simulink library "outp"  (R2021b)
settings: Solver=VariableStepAuto  StartTime=0.0  StopTime=10.0  RelTol=1e-3
undefined symbols (not defined in the file or in its folder): ENUM_PMMMODE_CHARGE, ENUM_PMMMODE_IDLE, ENUM_PMMMODE_INITIALIZE, ENUM_PMMMODE_POWERDOWN, ENUM_PMMMODE_SLEEP, Left, outp, slcm, TRUE
libraries: FVT_lib x736, hcu_lib x4, simulink x1
(part 4 of 8)

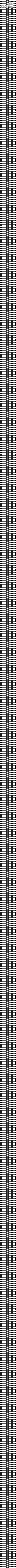
== system outp/OUTP/outpmodule ==
  VACC_HVTHCMSysAvail_enum : Inport
  VACC_LVBattVoltSta_enum : Inport  Port=2
  VACC_VehHVPwrAvail4THCM_W : Inport  Port=3
  VAPM_VehSpeed_kph : Inport  Port=4
  VAPM_VehSpeedTimeOut_flg : Inport  Port=5
  VAPM_FSOffSw_enum : Inport  Port=6
  VAPM_FSOffSwTimeOut_flg : Inport  Port=7
  VAPM_ChrgPlugSta_enum : Inport  Port=8
  VAPM_PASDRMR_cm : Inport  Port=9
  VAPM_PASDRML_cm : Inport  Port=10
  VAPM_PASDRCR_cm : Inport  Port=11
  VAPM_PASDRCL_cm : Inport  Port=12
  VAPM_PASDFMR_cm : Inport  Port=13
  VAPM_PASDFML_cm : Inport  Port=14
  VAPM_PASDFCR_cm : Inport  Port=15
  VAPM_PASDFCL_cm : Inport  Port=16
  VAPM_APSDRLR_cm : Inport  Port=17
  VAPM_APSDRLL_cm : Inport  Port=18
  VAPM_APSDFLR_cm : Inport  Port=19
  VAPM_APSDFLL_cm : Inport  Port=20
  VAPM_PASAFCL_enum : Inport  Port=21
  VAPM_PASARMR_enum : Inport  Port=22
  VAPM_PASARML_enum : Inport  Port=23
  VAPM_PASARCR_enum : Inport  Port=24
  VAPM_PASARCL_enum : Inport  Port=25
  VAPM_PASAFMR_enum : Inport  Port=26
  VAPM_PASAFML_enum : Inport  Port=27
  VAPM_PASAFCR_enum : Inport  Port=28
  VAPM_USSStaRMR_flg : Inport  Port=29
  VAPM_USSStaRML_flg : Inport  Port=30
  VAPM_USSStaRLR_flg : Inport  Port=31
  VAPM_USSStaRLL_flg : Inport  Port=32
  VAPM_USSStaRCR_flg : Inport  Port=33
  VAPM_USSStaRCL_flg : Inport  Port=34
  VAPM_USSStaFMR_flg : Inport  Port=35
  VAPM_USSStaFML_flg : Inport  Port=36
  VAPM_USSStaFLR_flg : Inport  Port=37
  VAPM_USSStaFLL_flg : Inport  Port=38
  VAPM_USSStaFCR_flg : Inport  Port=39
  VAPM_USSStaFCL_flg : Inport  Port=40
  VAPM_Chime_enum : Inport  Port=41
  VAPM_SNSRLayout_enum : Inport  Port=42
  VAPM_StaFSya_flg : Inport  Port=43
  VAPM_ModOperation_enum : Inport  Port=44
  VAPM_BrkPedalPos_pct : Inport  Port=45
  VAPM_BrkPedalPosTimeOut_flg : Inport  Port=46
  VAPM_LFRawWhlSpeed_kph : Inport  Port=47
  VAPM_LFRawWhlSpeedTimeOut_flg : Inport  Port=48
  VAPM_RFRawWhlSpeed_kph : Inport  Port=49
  VAPM_RFRawWhlSpeedTimeOut_flg : Inport  Port=50
  VAPM_LRRawWhlSpeed_kph : Inport  Port=51
  VAPM_LRRawWhlSpeedTimeOut_flg : Inport  Port=52
  VAPM_RRRawWhlSpeed_kph : Inport  Port=53
  VAPM_RRRawWhlSpeedTimeOut_flg : Inport  Port=54
  VAPM_LFRawWhlSpeedV_flg : Inport  Port=55
  VAPM_LFRawWhlSpeedVTimeOut_flg : Inport  Port=56
  VAPM_RFRawWhlSpeedV_flg : Inport  Port=57
  VAPM_RFRawWhlSpeedVTimeOut_flg : Inport  Port=58
  VAPM_LRRawWhlSpeedV_flg : Inport  Port=59
  VAPM_LRRawWhlSpeedVTimeOut_flg : Inport  Port=60
  VAPM_RRRawWhlSpeedV_flg : Inport  Port=61
  VAPM_RRRawWhlSpeedVTimeOut_flg : Inport  Port=62
  VAPM_LFWhlRotDir_enum : Inport  Port=63
  VAPM_LFWhlRotDirTimeOut_flg : Inport  Port=64
  VAPM_RFWhlRotDir_enum : Inport  Port=65
  VAPM_RFWhlRotDirTimeOut_flg : Inport  Port=66
  VAPM_LRWhlRotDir_enum : Inport  Port=67
  VAPM_LRWhlRotDirTimeOut_flg : Inport  Port=68
  VAPM_RRWhlRotDir_enum : Inport  Port=69
  VAPM_RRWhlRotDirTimeOut_flg : Inport  Port=70
  VAPM_LFPulseCountV_flg : Inport  Port=71
  VAPM_LFPulseCountVTimeOut_flg : Inport  Port=72
  VAPM_RFPulseCountV_flg : Inport  Port=73
  VAPM_RFPulseCountVTimeOut_flg : Inport  Port=74
  VAPM_LRPulseCountV_flg : Inport  Port=75
  VAPM_LRPulseCountVTimeOut_flg : Inport  Port=76
  VAPM_RRPulseCountV_flg : Inport  Port=77
  VAPM_RRPulseCountVTimeOut_flg : Inport  Port=78
  VAPM_LFPulseCount_enum : Inport  Port=79
  VAPM_LFPulseCountTimeOut_flg : Inport  Port=80
  VAPM_RFPulseCount_enum : Inport  Port=81
  VAPM_RFPulseCountTimeOut_flg : Inport  Port=82
  VAPM_LRPulseCount_enum : Inport  Port=83
  VAPM_LRPulseCountTimeOut_flg : Inport  Port=84
  VAPM_RRPulseCount_enum : Inport  Port=85
  VAPM_RRPulseCountTimeOut_flg : Inport  Port=86
  VAPM_ShifterHandleCmd_enum : Inport  Port=87
  VAPM_ShifterHandleCmdTimeOut_flg : Inport  Port=88
  VAPM_DriIntend_enum : Inport  Port=89
  VAPM_DriIntendTimeOut_flg : Inport  Port=90
  VAPM_EPSAOIControl_enum : Inport  Port=91
  VAPM_EPSAOIControlTimeOut_flg : Inport  Port=92
  VAPM_SASAngle_Deg : Inport  Port=93
  VAPM_SASAngleTimeOut_flg : Inport  Port=94
  VAPM_SASSpeed_degps : Inport  Port=95
  VAPM_SASSpeedTimeOut_flg : Inport  Port=96
  VAPM_SASSpeedValid_flg : Inport  Port=97
  VAPM_SASSpeedValidTimeOut_flg : Inport  Port=98
  VAPM_SASCAL_flg : Inport  Port=99
  VAPM_SASCALTimeOut_flg : Inport  Port=100
  VAPM_SASV_flg : Inport  Port=101
  VAPM_SASVTimeOut_flg : Inport  Port=102
  VAPM_GRADE_Deg : Inport  Port=103
  VAPM_GRADETimeOut_flg : Inport  Port=104
  VAPM_YawRate_degps : Inport  Port=105
  VAPM_YawRateTimeOut_flg : Inport  Port=106
  VAPM_LatAccel_Gps : Inport  Port=107
  VAPM_LatAccelTimeOut_flg : Inport  Port=108
  VAPM_LongAccel_Gps : Inport  Port=109
  VAPM_LongAccelTimeOut_flg : Inport  Port=110
  VAPM_MCPressure_bar : Inport  Port=111
  VAPM_MCPressureTimeOut_flg : Inport  Port=112
  VAPM_YawRateV_flg : Inport  Port=113
  VAPM_YawRateVTimeOut_flg : Inport  Port=114
  VAPM_LatAccelV_flg : Inport  Port=115
  VAPM_LatAccelVTimeOut_flg : Inport  Port=116
  VAPM_LongAccelV_flg : Inport  Port=117
  VAPM_LongAccelVTimeOut_flg : Inport  Port=118
  VAPM_MCPressureV_bar : Inport  Port=119
  VAPM_MCPressureVTimeOut_flg : Inport  Port=120
  VAPM_BrkSwSta_flg : Inport  Port=121
  VAPM_BrkSwStaTimeOut_flg : Inport  Port=122
  VAPM_BrkSwV_flg : Inport  Port=123
  VAPM_BrkSwVTimeOut_flg : Inport  Port=124
  VAPM_ESCStandstill_flg : Inport  Port=125
  VAPM_ESCStandstillTimeOut_flg : Inport  Port=126
  VAPM_ESCAPSSta_enum : Inport  Port=127
  VAPM_ESCAPSStaTimeOut_flg : Inport  Port=128
  VAPM_EPBExtReleaseAvail_flg : Inport  Port=129
  VAPM_EPBExtReleaseAvailTimeOut_flg : Inport  Port=130
  VAPM_EPBExtApplyAvail_flg : Inport  Port=131
  VAPM_EPBExtApplyAvailTimeOut_flg : Inport  Port=132
  VAPM_EPBErrSta_enum : Inport  Port=133
  VAPM_EPBErrStaTimeOut_flg : Inport  Port=134
  VAPM_EPBSta_enum : Inport  Port=135
  VAPM_EPBStaTimeOut_flg : Inport  Port=136
  VAPM_AVMparkingcancel_enum : Inport  Port=137
  VAPM_AVMparkingcancelTimeOut_flg : Inport  Port=138
  VAPM_AVMparkingexcute_enum : Inport  Port=139
  VAPM_AVMparkingexcuteTimeOut_flg : Inport  Port=140
  VAPM_AVMParkingmode_enum : Inport  Port=141
  VAPM_AVMParkingmodeTimeOut_flg : Inport  Port=142
  VAPM_AVMErrSTA_flg : Inport  Port=143
  VAPM_AVMErrSTATimeOut_flg : Inport  Port=144
  VAPM_IVIStatus_flg : Inport  Port=145
  VAPM_IVIStatusTimeOut_flg : Inport  Port=146
  VAPM_CAASSw_enum : Inport  Port=147
  VAPM_CAASSwTimeOut_flg : Inport  Port=148
  VAPM_IVIScreen_enum : Inport  Port=149
  VAPM_IVIScreenTimeOut_flg : Inport  Port=150
  VAPM_ABSActive_flg : Inport  Port=151
  VAPM_ABSActiveTimeOut_flg : Inport  Port=152
  VAPM_TCSActive_flg : Inport  Port=153
  VAPM_TCSActiveTimeOut_flg : Inport  Port=154
  VAPM_DriverSeatBeltCmd_flg : Inport  Port=155
  VAPM_DriverSeatBeltCmdTimeOut_flg : Inport  Port=156
  VAPM_APSProgressPCT_pct : Inport  Port=157
  VAPM_APSRQDisplay_enum : Inport  Port=158
  VAPM_APSSWVer_enum : Inport  Port=159
  VAPM_APSHWVer_enum : Inport  Port=160
  VAPM_APSExitCondition_enum : Inport  Port=161
  VAPM_APSAngleTarget_Deg : Inport  Port=162
  VAPM_APSVRqEPASCtrl_flg : Inport  Port=163
  VAPM_APSRqEPASCtrl_flg : Inport  Port=164
  VAPM_CAASSta_enum : Inport  Port=165
  VBCM_AntitheftSta_enum : Inport  Port=166
  VBCM_TailgateRemote_enum : Inport  Port=167
  VBCM_HornCtrl_flg : Inport  Port=168
  VBCM_AllDoorSW_flg : Inport  Port=169
  VBCM_BCMDoorLockSta_flg : Inport  Port=170
  VBCM_AntitheftSeatFlod_flg : Inport  Port=171
  VBCM_HoodSW_flg : Inport  Port=172
  VBCM_TailgateSW_flg : Inport  Port=173
  VBCM_DrDoorSW_flg : Inport  Port=174
  VBCM_PsDoorSW_flg : Inport  Port=175
  VBCM_RLDoorSW_flg : Inport  Port=176
  VBCM_RRDoorSW_flg : Inport  Port=177
  VBCM_LockSetting_flg : Inport  Port=178
  VBCM_FrChargingDoorCtrl_enum : Inport  Port=179
  VBCM_RrChargingDoorCtrl_enum : Inport  Port=180
  VBCM_CrashDetd_flg : Inport  Port=181
  VBCM_CTDCtrl_enum : Inport  Port=182
  VBCM_DoorLockIND_flg : Inport  Port=183
  VBCM_CTDLockSW_flg : Inport  Port=184
  VBCM_Dimmer_pct : Inport  Port=185
  VBCM_DimmerEN_flg : Inport  Port=186
  VBCM_PosLamp_flg : Inport  Port=187
  VBCM_LBeam_flg : Inport  Port=188
  VBCM_HBeam_flg : Inport  Port=189
  VBCM_RrFogLamp_flg : Inport  Port=190
  VBCM_BrakeLamp_flg : Inport  Port=191
  VBCM_ReverseLamp_flg : Inport  Port=192
  VBCM_LDRL_flg : Inport  Port=193
  VBCM_RDRL_flg : Inport  Port=194
  VBCM_LBSD_flg : Inport  Port=195
  VBCM_RBSD_flg : Inport  Port=196
  VBCM_HazardSW_flg : Inport  Port=197
  VBCM_LTurnLP_flg : Inport  Port=198
  VBCM_RTurnLP_flg : Inport  Port=199
  VBCM_BCMBuzzerReq_flg : Inport  Port=200
  VBCM_MirrorCtrl_enum : Inport  Port=201
  VBCM_MirrorDefog_flg : Inport  Port=202
  VBCM_RrDefog_flg : Inport  Port=203
  VBCM_RoomLampH_flg : Inport  Port=204
  VBCM_RoomLampL_flg : Inport  Port=205
  VBCM_TrunkRel_flg : Inport  Port=206
  VBCM_TailgateHDSW_flg : Inport  Port=207
  VBCM_FrWiperL_flg : Inport  Port=208
  VBCM_FrWiperH_flg : Inport  Port=209
  VBCM_RrWiper_flg : Inport  Port=210
  VBCM_WasherCtrl_enum : Inport  Port=211
  VBCM_WiperFixMode_flg : Inport  Port=212
  VBCM_User1DrAmbLightBrightness_enum : Inport  Port=213
  VBCM_User1IPAmbLightBrightness_enum : Inport  Port=214
  VBCM_User2DrAmbLightBrightness_enum : Inport  Port=215
  VBCM_User2IPAmbLightBrightness_enum : Inport  Port=216
  VBCM_User3DrAmbLightBrightness_enum : Inport  Port=217
  VBCM_User3IPAmbLightBrightness_enum : Inport  Port=218
  VBCM_User4DrAmbLightBrightness_enum : Inport  Port=219
  VBCM_User4IPAmbLightBrightness_enum : Inport  Port=220
  VBCM_User5DrAmbLightBrightness_enum : Inport  Port=221
  VBCM_User5IPAmbLightBrightness_enum : Inport  Port=222
  VBCM_User6DrAmbLightBrightness_enum : Inport  Port=223
  VBCM_User6IPAmbLightBrightness_enum : Inport  Port=224
  VBCM_User1AmbLightColor_enum : Inport  Port=225
  VBCM_User2AmbLightColor_enum : Inport  Port=226
  VBCM_User3AmbLightColor_enum : Inport  Port=227
  VBCM_User4AmbLightColor_enum : Inport  Port=228
  VBCM_User5AmbLightColor_enum : Inport  Port=229
  VBCM_User6AmbLightColor_enum : Inport  Port=230
  VBCM_AmbLightBreath1_flg : Inport  Port=231
  VBCM_AmbLightBreath2_flg : Inport  Port=232
  VBCM_AmbLightBreath3_flg : Inport  Port=233
  VBCM_AmbLightBrightness1_enum : Inport  Port=234
  VBCM_AmbLightBrightness2_enum : Inport  Port=235
  VBCM_AmbLightBrightness3_enum : Inport  Port=236
  VBCM_AmbLightColor1_enum : Inport  Port=237
  VBCM_AmbLightColor2_enum : Inport  Port=238
  VBCM_AmbLightColor3_enum : Inport  Port=239
  VBCM_LampPwr_flg : Inport  Port=240
  VBCM_SPTGDet_flg : Inport  Port=241
  VBCM_APSOpenPTG_flg : Inport  Port=242
  VBCM_FollowMe_flg : Inport  Port=243
  VBCM_IVIRST_flg : Inport  Port=244
  VBCM_CountAlarm_enum : Inport  Port=245
  VBCM_MFSWTri_flg : Inport  Port=246
  VBCM_MirrorFlodPos_flg : Inport  Port=247
  VBCM_FuelDoorPos_flg : Inport  Port=248
  VBCM_MFRDNBrightReq_pct : Inport  Port=249
  VBCM_RoomLampMode_flg : Inport  Port=250
  VBCM_IVIPTGUSStaSW_flg : Inport  Port=251
  VBCM_PTGInnerSW2_enum : Inport  Port=252
  VBCM_LDrvCtrlCmd_pct : Inport  Port=253
  VBCM_LPasCtrlCmd_pct : Inport  Port=254
  VBCM_LRLDCtrlCmd_pct : Inport  Port=255
  VBCM_LRRDCtrlCmd_pct : Inport  Port=256
  VBCM_APMDoorControlSta_flg : Inport  Port=257
  VBCM_LockAlarm_enum : Inport  Port=258
  VBCM_ATCtrl_enum : Inport  Port=259
  VBCM_fUnlockSingle_flg : Inport  Port=260
  VBCM_OutMode_enum : Inport  Port=261
  VDDM_C3BMS6RCDTC_raw32 : Inport  Port=262
  VDDM_C3BMS6CSDTC_raw32 : Inport  Port=263
  VDDM_C3BMS6LCDTC_raw32 : Inport  Port=264
  VDDM_C3BMS1RCDTC_raw32 : Inport  Port=265
  VDDM_C3BMS1CSDTC_raw32 : Inport  Port=266
  VDDM_C3BMS1LCDTC_raw32 : Inport  Port=267
  VDDM_C3CCU1RCDTC_raw32 : Inport  Port=268
  VDDM_C3CCU1CSDTC_raw32 : Inport  Port=269
  VDDM_C3CCU1LCDTC_raw32 : Inport  Port=270
  VDDM_C3CCU2RCDTC_raw32 : Inport  Port=271
  VDDM_C3CCU2CSDTC_raw32 : Inport  Port=272
  VDDM_C3CCU2LCDTC_raw32 : Inport  Port=273
  VDDM_C1ABM1RCDTC_raw32 : Inport  Port=274
  VDDM_C1ABM1CSDTC_raw32 : Inport  Port=275
  VDDM_C1ABM1LCDTC_raw32 : Inport  Port=276
  VDDM_Lv1ErrDTC_raw32 : Inport  Port=277
  VDDM_Lv2ErrDTC_raw32 : Inport  Port=278
  VDDM_Lv3ErrDTC_raw32 : Inport  Port=279
  VDDM_Lv4ErrDTC_raw32 : Inport  Port=280
  VDDM_BrkSWErrDTC_raw32 : Inport  Port=281
  VDDM_BrkSWNoBacDTC_raw32 : Inport  Port=282
  VDDM_KeyAuthDTC_raw32 : Inport  Port=283
  VDDM_ONtoRdyDTC_raw32 : Inport  Port=284
  VDDM_HVB4PreDTC_raw32 : Inport  Port=285
  VDDM_MCU4PreDTC_raw32 : Inport  Port=286
  VDDM_DCDC4PreDTC_raw32 : Inport  Port=287
  VDDM_HVRlyCloDTC_raw32 : Inport  Port=288
  VDDM_BMSRdyDTC_raw32 : Inport  Port=289
  VDDM_DCDCEnaDTC_raw32 : Inport  Port=290
  VDDM_HiLvSaChkDTC_raw32 : Inport  Port=291
  VDDM_MidLvSaChkDTC_raw32 : Inport  Port=292
  VDDM_MCUDisDTC_raw32 : Inport  Port=293
  VDDM_DCDCDisDTC_raw32 : Inport  Port=294
  VDDM_HVRlyOpDTC_raw32 : Inport  Port=295
  VDDM_MCUActDTC_raw32 : Inport  Port=296
  VDDM_OBC4PreDTC_raw32 : Inport  Port=297
  VDDM_IniLVLoDTC_raw32 : Inport  Port=298
  VDDM_LVSupLoDTC_raw32 : Inport  Port=299
  VDDM_LVSupHiDTC_raw32 : Inport  Port=300
  VDDM_DrStSWDTC_raw32 : Inport  Port=301
  VDDM_FLDoorSWDTC_raw32 : Inport  Port=302
  VDDM_RLDoorSWDTC_raw32 : Inport  Port=303
  VDDM_FRDoorSWDTC_raw32 : Inport  Port=304
  VDDM_RRDoorSWDTC_raw32 : Inport  Port=305
  VDDM_HoodSWDTC_raw32 : Inport  Port=306
  VDDM_TailgaSWDTC_raw32 : Inport  Port=307
  VDDM_VehMalfunLevel_enum : Inport  Port=308
  VDDM_APS1SigOoRDTC_raw32 : Inport  Port=309
  VDDM_APS2SigOoRDTC_raw32 : Inport  Port=310
  VDDM_APSCorrErrDTC_raw32 : Inport  Port=311
  VDDM_MCUF1NoComDTC_raw32 : Inport  Port=312
  VDDM_MCUR1NoComDTC_raw32 : Inport  Port=313
  VDDM_Shifter1NoComDTC_raw32 : Inport  Port=314
  VDDM_ESC7NoComDTC_raw32 : Inport  Port=315
  VDDM_ESC1NoComDTC_raw32 : Inport  Port=316
  VDDM_ESC5NoComDTC_raw32 : Inport  Port=317
  VDDM_EnterNewOperCyc_flg : Inport  Port=318
  VDDM_DiagHCrashDTC_raw32 : Inport  Port=319
  VDDM_DiagFLTSDTC_raw32 : Inport  Port=320
  VDDM_DiagFRTSDTC_raw32 : Inport  Port=321
  VDDM_DiagRLTSDTC_raw32 : Inport  Port=322
  VDDM_DiagRRTSDTC_raw32 : Inport  Port=323
  VDDM_FCLUSSDTC_raw32 : Inport  Port=324
  VDDM_FMLUSSDTC_raw32 : Inport  Port=325
  VDDM_FMRUSSDTC_raw32 : Inport  Port=326
  VDDM_FCRUSSDTC_raw32 : Inport  Port=327
  VDDM_RCLUSSDTC_raw32 : Inport  Port=328
  VDDM_RMLUSSDTC_raw32 : Inport  Port=329
  VDDM_RMRUSSDTC_raw32 : Inport  Port=330
  VDDM_RCRUSSDTC_raw32 : Inport  Port=331
  VDDM_FLLUSSDTC_raw32 : Inport  Port=332
  VDDM_FLRUSSDTC_raw32 : Inport  Port=333
  VDDM_RLLUSSDTC_raw32 : Inport  Port=334
  VDDM_RLRUSSDTC_raw32 : Inport  Port=335
  VDDM_FCM2NoComDTC_raw32 : Inport  Port=336
  VDDM_FCM2RCErrDTC_raw32 : Inport  Port=337
  VDDM_FCM2CSErrDTC_raw32 : Inport  Port=338
  VDDM_FCM3NoComDTC_raw32 : Inport  Port=339
  VDDM_FCM3RCErrDTC_raw32 : Inport  Port=340
  VDDM_FCM3CSErrDTC_raw32 : Inport  Port=341
  VDDM_FCM4NoComDTC_raw32 : Inport  Port=342
  VDDM_FCM4CSErrDTC_raw32 : Inport  Port=343
  VDDM_FCM5NoComDTC_raw32 : Inport  Port=344
  VDDM_FCM5CSErrDTC_raw32 : Inport  Port=345
  VDDM_ZoneSCPNoComDTC_raw32 : Inport  Port=346
  VDDM_BMSSigErrDetDTC_raw32 : Inport  Port=347
  VDDM_FCMACCSigErrDetDTC_raw32 : Inport  Port=348
  VDDM_FrMCUSigErrDetDTC_raw32 : Inport  Port=349
  VDDM_RrMCUSigErrDetDTC_raw32 : Inport  Port=350
  VDDM_CCUSigErrDetDTC_raw32 : Inport  Port=351
  VDDM_ACCAccelCmdErrDetDTC_raw32 : Inport  Port=352
  VDDM_ACCMalfuncDetDTC_raw32 : Inport  Port=353
  VDDM_CCMalfuncDetDTC_raw32 : Inport  Port=354
  VDDM_MSAMalfuncDetDTC_raw32 : Inport  Port=355
  VDDM_ISAMalfuncDetDTC_raw32 : Inport  Port=356
  VDDM_MCUF1RCErrDTC_raw32 : Inport  Port=357
  VDDM_MCUR1RCErrDTC_raw32 : Inport  Port=358
  VDDM_MCUF1CSErrDTC_raw32 : Inport  Port=359
  VDDM_MCUR1CSErrDTC_raw32 : Inport  Port=360
  VDDM_Shifter1RCErrDTC_raw32 : Inport  Port=361
  VDDM_Shifter1CSErrDTC_raw32 : Inport  Port=362
  VDDM_ESC7RCErrDTC_raw32 : Inport  Port=363
  VDDM_ESC7CSErrDTC_raw32 : Inport  Port=364
  VDDM_ESC1RCErrDTC_raw32 : Inport  Port=365
  VDDM_ESC1CSErrDTC_raw32 : Inport  Port=366
  VDDM_ESC5RCErrDTC_raw32 : Inport  Port=367
  VDDM_ESC5CSErrDTC_raw32 : Inport  Port=368
  VDDM_FrMCUTqErrDTC_raw32 : Inport  Port=369
  VDDM_RrMCUTqErrDTC_raw32 : Inport  Port=370
  VDDM_LFBatwarnDTC_raw32 : Inport  Port=371
  VDDM_RFBatwarnDTC_raw32 : Inport  Port=372
  VDDM_LRBatwarnDTC_raw32 : Inport  Port=373
  VDDM_RRBatwarnDTC_raw32 : Inport  Port=374
  VDDM_LFPressIndiDTC_raw32 : Inport  Port=375
  VDDM_RFPressIndiDTC_raw32 : Inport  Port=376
  VDDM_LRPressIndiDTC_raw32 : Inport  Port=377
  VDDM_RRPressIndiDTC_raw32 : Inport  Port=378
  VDDM_LFWheelTmpHighDTC_raw32 : Inport  Port=379
  VDDM_RFWheelTmpHighDTC_raw32 : Inport  Port=380
  VDDM_LRWheelTmpHighDTC_raw32 : Inport  Port=381
  VDDM_RRWheelTmpHighDTC_raw32 : Inport  Port=382
  VDDM_LFSensorFailDTC_raw32 : Inport  Port=383
  VDDM_RFSensorFailDTC_raw32 : Inport  Port=384
  VDDM_LRSensorFailDTC_raw32 : Inport  Port=385
  VDDM_RRSensorFailDTC_raw32 : Inport  Port=386
  VDDM_C1EPAS2LCDTC_raw32 : Inport  Port=387
  VDDM_5vAPS1PwrErrDTC_raw32 : Inport  Port=388
  VDDM_5vAPS2PwrErrDTC_raw32 : Inport  Port=389
  VDDM_EPBLockTODTC_raw32 : Inport  Port=390
  VDDM_EPBUnlockTODTC_raw32 : Inport  Port=391
  VDDM_THCMAPTCWarning_raw32 : Inport  Port=392
  VDDM_LimpHomeActTmp_flg : Inport  Port=393
  VDDM_EDriveSysErr_VCUErrTmp_flg : Inport  Port=394
  VDHP_ActAPSPosn_pct : Inport  Port=395
  VDHP_EAPS1MIN_pct : Inport  Port=396
  VDHP_EAPS2MIN_pct : Inport  Port=397
  VDKC_DKCTimeSN_cnt : Inport  Port=398
  VDKC_DKCAuthSta_enum : Inport  Port=399
  VNMM_AllCANTxReq_flg : Inport  Port=400
  VNMM_NMmTxReq_flg : Inport  Port=401
  VNMM_Awake_enum : Inport  Port=402
  VNMM_CSB_flg : Inport  Port=403
  VNMM_ErrorState_enum : Inport  Port=404
  VNMM_NodeID_enum : Inport  Port=405
  VNMM_PNI_flg : Inport  Port=406
  VNMM_RptMsgReq_flg : Inport  Port=407
  VNMM_WakeUp_enum : Inport  Port=408
  VNMM_ActiveWU_flg : Inport  Port=409
  VNMM_SysNMmSta_enum : Inport  Port=410
  VNMM_NetworkReq_flg : Inport  Port=411
  VPMM_PowerUpState_enum : Inport  Port=412
  VPMM_PowerDownState_enum : Inport  Port=413
  VPMM_PowerUpFault_enum : Inport  Port=414
  VPMM_PowerDownFault_enum : Inport  Port=415
  VPMM_ActiveDischargeReq_flg : Inport  Port=416
  VPMM_DCDCEnaReq_flg : Inport  Port=417
  VPMM_DCDCVoltSetpoint_V : Inport  Port=418
  VPMM_HVBatCnctReq_flg : Inport  Port=419
  VPMM_HVSysReadyToCharge_enum : Inport  Port=420
  VPMM_PowerSta_enum : Inport  Port=421
  VPMM_LVPwrSta_flg : Inport  Port=422
  VPMM_HVPwrSta_flg : Inport  Port=423
  VPMM_SysPowerMode_enum : Inport  Port=424
  VPMM_FrMCUEnaReq_flg : Inport  Port=425
  VPMM_RrMCUEnaReq_flg : Inport  Port=426
  VPMM_DrivetrainSelect_enum : Inport  Port=427
  VPMM_DrSeatSta_enum : Inport  Port=428
  VPMM_PwrStaSelect_enum : Inport  Port=429
  VPMM_PwrStaConstraint_enum : Inport  Port=430
  VPMM_TCountSta_enum : Inport  Port=431
  VPMM_PwrUpReq_enum : Inport  Port=432
  VPMM_PwrDownReq_enum : Inport  Port=433
  VPMM_LowSOCWarn_enum : Inport  Port=434
  VPMM_ReVehThdChkSta_enum : Inport  Port=435
  VPMM_LVSysErrPwrOutErr_flg : Inport  Port=436
  VPMM_EvccAplusPwrUpReq_flg : Inport  Port=437
  VPMM_PwrStaONTOPopReq_flg : Inport  Port=438
  VPMM_IVIPwrStaONTOPopT_s : Inport  Port=439
  VPMM_LVChrgHoldTtimer_s : Inport  Port=440
  VPMM_LVBattChrgTimeCnt_s : Inport  Port=441
  VPMM_SilentChkAllowSleep_flg : Inport  Port=442
  VPMM_TimerAllowSleep_flg : Inport  Port=443
  VPMM_FDADC12VDetAvg_mV : Inport  Port=444
  VPMM_PMMAllowECUSleep_flg : Inport  Port=445
  VPMM_LVSilentChrgSta_enum : Inport  Port=446
  VPMM_LVSilentChrgReq_flg : Inport  Port=447
  VPMM_LVSilentChrgLv_enum : Inport  Port=448
  VPMM_CtrlFrPwrStbA1P_flg : Inport  Port=449
  VPMM_CtrlFrRC1_flg : Inport  Port=450
  VPMM_CtrlFrBMSCCUCIR_flg : Inport  Port=451
  VPMM_CtrlFrEDUINVERTER_flg : Inport  Port=452
  VPMM_HWResetSta_enum : Inport  Port=453
  VPMM_CtrlDrPwrStbA2_flg : Inport  Port=454
  VPMM_PwrStaTOSta_enum : Inport  Port=455
  VPMM_Sched_ChgTOSta_enum : Inport  Port=456
  VPMM_PwrReq_OTA_enum : Inport  Port=457
  VPMM_OTAPwrReqOFFChkSta_enum : Inport  Port=458
  VPMM_OTAPwrReqStdChkSta_enum : Inport  Port=459
  VSYS_HWVer1_cnt : Inport  Port=460
  VSYS_HWVer2_cnt : Inport  Port=461
  VSYS_HWVer3_cnt : Inport  Port=462
  VSYS_CarModel1_cnt : Inport  Port=463
  VSYS_CarModel2_cnt : Inport  Port=464
  VSYS_CarModel3_cnt : Inport  Port=465
  VSYS_ECU1_cnt : Inport  Port=466
  VSYS_ECU2_cnt : Inport  Port=467
  VSYS_Major1_cnt : Inport  Port=468
  VSYS_Major2_cnt : Inport  Port=469
  VSYS_Minor1_cnt : Inport  Port=470
  VSYS_Minor2_cnt : Inport  Port=471
  VSYS_Patch1_cnt : Inport  Port=472
  VSYS_Patch2_cnt : Inport  Port=473
  VSYS_Country1_cnt : Inport  Port=474
  VSYS_Country2_cnt : Inport  Port=475
  VSYS_Variation_cnt : Inport  Port=476
  VSYS_Dash1_cnt : Inport  Port=477
  VSYS_Change1_cnt : Inport  Port=478
  VSYS_Change2_cnt : Inport  Port=479
  VSYS_Dash2_cnt : Inport  Port=480
  VSYS_SHA1_cnt : Inport  Port=481
  VSYS_SHA2_cnt : Inport  Port=482
  VSYS_SHA3_cnt : Inport  Port=483
  VSYS_SHA4_cnt : Inport  Port=484
  VSYS_SHA5_cnt : Inport  Port=485
  VSYS_SHA6_cnt : Inport  Port=486
  VSYS_SHA7_cnt : Inport  Port=487
  VSYS_SHA8_cnt : Inport  Port=488
  VSYS_NvWriteReqRisingEdge_flg : Inport  Port=489
  VSYS_FdcSlpReqRisingEdge_flg : Inport  Port=490
  VSYS_FdcSlpTime_sec : Inport  Port=491
  VSYS_PmicBootReason_enum : Inport  Port=492
  VSYS_WisrBootReason_raw32 : Inport  Port=493
  VSYS_AcoreRebootCmdACK_flg : Inport  Port=494
  VSYS_CurrentNmState_enum : Inport  Port=495
  VTHC_FDCompCmd_rpm : Inport  Port=496
  VTHC_FDSOV1Cmd_flg : Inport  Port=497
  VTHC_FDSOV2Cmd_flg : Inport  Port=498
  VTHC_FDSOV3Cmd_flg : Inport  Port=499
  VTHC_FDEXV1Cmd_step : Inport  Port=500
  VTHC_FDEXV2Cmd_step : Inport  Port=501
  VTHC_FDSOTXVCmd_flg : Inport  Port=502
  VTHC_FDFWVCmd_flg : Inport  Port=503
  VTHC_FDTWVCmd_pct : Inport  Port=504
  VTHC_FDFrWPTCHeatPwrCmd_W : Inport  Port=505
  VTHC_CoolgFanActDuty_pct : Inport  Port=506
  VTHC_FDAGSCmd_enum : Inport  Port=507
  VTHC_FDEWP1Cmd_enum : Inport  Port=508
  VTHC_FDEWP2Cmd_enum : Inport  Port=509
  VTHC_FDEWP3Cmd_enum : Inport  Port=510
  VTHC_FDFrLeAPTCHeatPwrCmd_W : Inport  Port=511
  VTHC_FDFrRiAPTCHeatPwrCmd_W : Inport  Port=512
  VTHC_FDRrAPTCHeatPwrCmd_W : Inport  Port=513
  VTHC_FDBlowerCmd_pct : Inport  Port=514
  VTHC_BatteryMode_enum : Inport  Port=515
  VTHC_EDriveMode_enum : Inport  Port=516
  VTHC_CabinMode_enum : Inport  Port=517
  VTHC_CCUACLampSts_flg : Inport  Port=518
  VTHC_CCUAutoLampSts_flg : Inport  Port=519
  VTHC_CCUACMaxLampSts_flg : Inport  Port=520
  VTHC_CCUSyncLampSts_flg : Inport  Port=521
  VTHC_sigAirIntenZon1St_enum : Inport  Port=522
  VTHC_sigWindDirZon1St_enum : Inport  Port=523
  VTHC_sigRecircSt_flg : Inport  Port=524
  VTHC_sigSetTempZon1St_C : Inport  Port=525
  VTHC_sigSetTempZon2St_C : Inport  Port=526
  VTHC_sigClntTHvBattOut_C : Inport  Port=527
  VTHC_sigCbnSolarLeft_W : Inport  Port=528
  VTHC_sigClntTHvBattIn_C : Inport  Port=529
  VTHC_sigCbnSolarRight_W : Inport  Port=530
  VTHC_sigAmbAirT_C : Inport  Port=531
  VTHC_sigCbnAirT_C : Inport  Port=532
  VTHC_ACSubMode_enum : Inport  Port=533
  VTHC_FDRecyAutoCmd_enum : Inport  Port=534
  VTHC_ACModeMem_enum : Inport  Port=535
  VTHC_Face_flg : Inport  Port=536
  VTHC_Foot_flg : Inport  Port=537
  VTHC_Frost_flg : Inport  Port=538
  VTHC_FaceM_flg : Inport  Port=539
  VTHC_FootM_flg : Inport  Port=540
  VTHC_CCUSyncSts_flg : Inport  Port=541
  VTHC_ACForceOFF_flg : Inport  Port=542
  VTHC_RecAutoFlg_flg : Inport  Port=543
  VTHC_AirIntenZone1M_enum : Inport  Port=544
  VTHC_fdefog_flg : Inport  Port=545
  VTHC_sigSetTempZon2StM_C : Inport  Port=546
  VTHC_sigDfrstSt_flg : Inport  Port=547
  VTHC_FDCTHCAirIntZ3Sta_enum : Inport  Port=548
  VTHC_FDCTHCDrEVentModeSta_enum : Inport  Port=549
  VTHC_FDCTHCPsEVentModeSta_enum : Inport  Port=550
  VTHC_FDCTHCDrEVentZSta_enum : Inport  Port=551
  VTHC_FDCTHCCLEVentZSta_enum : Inport  Port=552
  VTHC_FDCTHCPsEVentZSta_enum : Inport  Port=553
  VTHC_FDCTHCCREVentZSta_enum : Inport  Port=554
  VTHC_FDCTHCDrEVentYSta_enum : Inport  Port=555
  VTHC_FDCTHCDrVentENSta_flg : Inport  Port=556
  VTHC_FDCTHCCLEVentYSta_enum : Inport  Port=557
  VTHC_FDCTHCCLVentENSta_flg : Inport  Port=558
  VTHC_FDCTHCPsEVentYSta_enum : Inport  Port=559
  VTHC_FDCTHCPsVentENSta_flg : Inport  Port=560
  VTHC_FDCTHCCREVentYSta_enum : Inport  Port=561
  VTHC_FDCTHCCRVentENSta_flg : Inport  Port=562
  VTHC_FDCTHCMAPTCForceOFFSta_flg : Inport  Port=563
  VTHC_DrVentEN_flg : Inport  Port=564
  VTHC_CLVentEN_flg : Inport  Port=565
  VTHC_PsVentEN_flg : Inport  Port=566
  VTHC_CRVentEN_flg : Inport  Port=567
  VTHC_FDCFGSAirIntSta_enum : Inport  Port=568
  VTHC_FDCFGSChSta_enum : Inport  Port=569
  VTHC_FDCFGSAirIntCmd_enum : Inport  Port=570
  VTHC_FDCFGSFuncSta_flg : Inport  Port=571
  VTHC_FDCFGSChCmd_enum : Inport  Port=572
  VTHC_FDCFGSIONSWSta_flg : Inport  Port=573
  VTHC_FDCFGSIONCmd_flg : Inport  Port=574
  VTHC_FDCFGSLearnCmd_enum : Inport  Port=575
  VTHC_FDCTHCMPreWPTCHeatSta_enum : Inport  Port=576
  VTPM_LFBatWarn_flg : Inport  Port=577
  VTPM_RFBatWarn_flg : Inport  Port=578
  VTPM_LRBatWarn_flg : Inport  Port=579
  VTPM_RRBatWarn_flg : Inport  Port=580
  VTPM_LFWheelPress_raw8 : Inport  Port=581
  VTPM_RFWheelPress_raw8 : Inport  Port=582
  VTPM_LRWheelPress_raw8 : Inport  Port=583
  VTPM_RRWheelPress_raw8 : Inport  Port=584
  VTPM_LFWheelTemp_C : Inport  Port=585
  VTPM_RFWheelTemp_C : Inport  Port=586
  VTPM_LRWheelTemp_C : Inport  Port=587
  VTPM_RRWheelTemp_C : Inport  Port=588
  VTPM_LFSensorFail_flg : Inport  Port=589
  VTPM_RFSensorFail_flg : Inport  Port=590
  VTPM_LRSensorFail_flg : Inport  Port=591
  VTPM_RRSensorFail_flg : Inport  Port=592
  VTPM_LFWheelDebug_flg : Inport  Port=593
  VTPM_LRWheelDebug_flg : Inport  Port=594
  VTPM_RFWheelDebug_flg : Inport  Port=595
  VTPM_RRWheelDebug_flg : Inport  Port=596
  VTPM_TPMSResButtAllow_flg : Inport  Port=597
  VTPM_TPMSCaliButtAllow_flg : Inport  Port=598
  VTPM_LFPressIndi_enum : Inport  Port=599
  VTPM_RFPressIndi_enum : Inport  Port=600
  VTPM_LRPressIndi_enum : Inport  Port=601
  VTPM_RRPressIndi_enum : Inport  Port=602
  VTPM_TPMSWarnIndi_enum : Inport  Port=603
  VTPM_LFWheelTmpIndi_flg : Inport  Port=604
  VTPM_RFWheelTmpIndi_flg : Inport  Port=605
  VTPM_LRWheelTmpIndi_flg : Inport  Port=606
  VTPM_RRWheelTmpIndi_flg : Inport  Port=607
  VTPM_LFWheelPSW_raw8 : Inport  Port=608
  VTPM_LRWheelPSW_raw8 : Inport  Port=609
  VTPM_RFWheelPSW_raw8 : Inport  Port=610
  VTPM_RRWheelPSW_raw8 : Inport  Port=611
  VTPM_CWheelTips_enum : Inport  Port=612
  VTPM_AutoLTips_enum : Inport  Port=613
  VTPM_LFSensorMode_flg : Inport  Port=614
  VTPM_RFSensorMode_flg : Inport  Port=615
  VTPM_LRSensorMode_flg : Inport  Port=616
  VTPM_RRSensorMode_flg : Inport  Port=617
  VTPM_S1ID_raw32 : Inport  Port=618
  VTPM_S2ID_raw32 : Inport  Port=619
  VTPM_S3ID_raw32 : Inport  Port=620
  VTPM_S4ID_raw32 : Inport  Port=621
  VTPM_S1L_enum : Inport  Port=622
  VTPM_S2L_enum : Inport  Port=623
  VTPM_S3L_enum : Inport  Port=624
  VTPM_S4L_enum : Inport  Port=625
  VTPM_ALFin_flg : Inport  Port=626
  VTPM_LFP20_raw8 : Inport  Port=627
  VTPM_RFP20_raw8 : Inport  Port=628
  VTPM_LRP20_raw8 : Inport  Port=629
  VTPM_RRP20_raw8 : Inport  Port=630
  VTPM_FAT_flg : Inport  Port=631
  VTPM_IDin_raw32 : Inport  Port=632
  VTPM_S1WheelDebugALTU_pct : Inport  Port=633
  VTPM_S2WheelDebugALTU_pct : Inport  Port=634
  VTPM_S3WheelDebugALTU_pct : Inport  Port=635
  VTPM_S4WheelDebugALTU_pct : Inport  Port=636
  VTPM_ID1messageALTU_raw8 : Inport  Port=637
  VTPM_ID2messageALTU_raw8 : Inport  Port=638
  VTPM_ID3messageALTU_raw8 : Inport  Port=639
  VTPM_ID4messageALTU_raw8 : Inport  Port=640
  VTPM_Chkfin_flg : Inport  Port=641
  VTPM_SetIDLoc_flg : Inport  Port=642
  VTPM_TPMSStorge_flg : Inport  Port=643
  VTPM_ChkStorge_flg : Inport  Port=644
  VTPM_TPMSResButt_flg : Inport  Port=645
  VTPM_LFPindi_enum : Inport  Port=646
  VTPM_RFPind_enum : Inport  Port=647
  VTPM_LRPindi_enum : Inport  Port=648
  VTPM_RRPindi_enum : Inport  Port=649
  VTPM_WriteChkLFID_raw : Inport  Port=650
  VTPM_WriteChkRFID_raw : Inport  Port=651
  VTPM_WriteChkLRID_raw : Inport  Port=652
  VTPM_WriteChkRRID_raw : Inport  Port=653
  VTPM_WriteChkfinLFID_raw : Inport  Port=654
  VTPM_WriteChkfinRFID_raw : Inport  Port=655
  VTPM_WriteChkfinLRID_raw : Inport  Port=656
  VTPM_WriteChkfinRRID_raw : Inport  Port=657
  VTPM_Flashchkdatavalid_enum : Inport  Port=658
  VTPM_Flashdatavalid_enum : Inport  Port=659
  VTPM_unlearnSfali_flg : Inport  Port=660
  VTPM_unlearnSfailvalid_enum : Inport  Port=661
  VTPM_Prepresstempvalid_enum : Inport  Port=662
  VTPM_FlashS1ID_raw : Inport  Port=663
  VTPM_FlashS2ID_raw : Inport  Port=664
  VTPM_FlashS3ID_raw : Inport  Port=665
  VTPM_FlashS4ID_raw : Inport  Port=666
  VTPM_FlashIDvalid_enum : Inport  Port=667
  VTPM_WritingCnt_enum : Inport  Port=668
  VTPM_TPMSTLCmd_flg : Inport  Port=669
  VTPM_LProgress_enum : Inport  Port=670
  VTPM_TPMSSensorIDRegStart_flg : Inport  Port=671
  VTPM_ModelVersion_raw : Inport  Port=672
  VTPM_ModelVersionChksum_raw : Inport  Port=673
  VTQD_ParkRequest_flg : Inport  Port=674
  VTQD_TqSourceFr_enum : Inport  Port=675
  VTQD_TqSourceRr_enum : Inport  Port=676
  VTQD_FrEDUAvailBrkRgnTq_Nm : Inport  Port=677
  VTQD_RrEDUAvailBrkRgnTq_Nm : Inport  Port=678
  VTQD_EVDriveMode_enum : Inport  Port=679
  VTQD_ShiftGearPosn_enum : Inport  Port=680
  VTQD_PButtonSta_enum : Inport  Port=681
  VTQD_FrActvDmpDisabReq_flg : Inport  Port=682
  VTQD_RrActvDmpDisabReq_flg : Inport  Port=683
  VTQD_FrRgnDecrSta_flg : Inport  Port=684
  VTQD_RrRgnDecrSta_flg : Inport  Port=685
  VTQD_DriverWhlTqDemFr_Nm : Inport  Port=686
  VTQD_DriverWhlTqDemRr_Nm : Inport  Port=687
  VTQD_FrEDUActTq_Nm : Inport  Port=688
  VTQD_RrEDUActTq_Nm : Inport  Port=689
  VTQD_FrEDURolRgnTq_Nm : Inport  Port=690
  VTQD_RrEDURolRgnTq_Nm : Inport  Port=691
  VTQD_FrEDUSpd_rpm : Inport  Port=692
  VTQD_RrEDUSpd_rpm : Inport  Port=693
  VTQD_FrEDUSpdValid_flg : Inport  Port=694
  VTQD_FrEDUAvailBrkRgnTqV_flg : Inport  Port=695
  VTQD_RrEDUSpdValid_flg : Inport  Port=696
  VTQD_RrEDUAvailBrkRgnTqV_flg : Inport  Port=697
  VTQD_RgnAbnorSta_flg : Inport  Port=698
  VTQD_PTCSPermSta_flg : Inport  Port=699
  VTQD_FrRgnPermSta_flg : Inport  Port=700
  VTQD_RrRgnPermSta_flg : Inport  Port=701
  VTQD_FrIdcMin_A : Inport  Port=702
  VTQD_FrIdcMax_A : Inport  Port=703
  VTQD_FrUdcMin_V : Inport  Port=704
  VTQD_FrUdcMax_V : Inport  Port=705
  VTQD_RrIdcMin_A : Inport  Port=706
  VTQD_RrIdcMax_A : Inport  Port=707
  VTQD_RrUdcMin_V : Inport  Port=708
  VTQD_RrUdcMax_V : Inport  Port=709
  VTQD_ReBrakeLPReq_flg : Inport  Port=710
  VTQD_CreepON_flg : Inport  Port=711
  VTQD_EquivAccPedalSWSta_flg : Inport  Port=712
  VTQD_DriveProtEn_flg : Inport  Port=713
  VTQD_ActParkRequest_flg : Inport  Port=714
  VTQD_IVIPwrLockSta_enum : Inport  Port=715
  VTQD_OPDHoldLamp_flg : Inport  Port=716
  VTQD_VehActSpd_kph : Inport  Port=717
  VTQR_FrTMTqReq_Nm : Inport  Port=718
  VTQR_RrTMTqReq_Nm : Inport  Port=719
  VV2L_ReqOBCV2LEna_enum : Inport  Port=720
  VV2L_ReqV2LIVIPopup_enum : Inport  Port=721
  VVMC_ACCCtrlAvail_flg : Inport  Port=722
  VVMC_ACCPedalOvrd_flg : Inport  Port=723
  VVMC_CCCtrlSta_enum : Inport  Port=724
  VVMC_CCMSASpdWar_flg : Inport  Port=725
  VVMC_MSACtrlSta_enum : Inport  Port=726
  VVMC_APSCtrlAvail_flg : Inport  Port=727
  VVMC_APSActive_flg : Inport  Port=728
  VVMC_APSStaSys_enum : Inport  Port=729
  VVMC_APSDecReqA_flg : Inport  Port=730
  VVMC_APSDecReq_mps2 : Inport  Port=731
  VVMC_APSReq_enum : Inport  Port=732
  VVMC_IMUEnaCmd_flg : Inport  Port=733
  VVMC_CAASCtrlAvail_flg : Inport  Port=734
  VVMC_CAASActive_flg : Inport  Port=735
  VVMC_ExtraMSACtrlSta_enum : Inport  Port=736
  UnitConverter{1..2,6,8..16,21..28,41..42,44,63,65,67,69,79,81,83,85,87,89,91,127,133,135,137,139,141,147,149,158..161,165..167,179..180,182,201,211,213..230,234..239,245,249,252..256,258..259,261,308,399,402,404..405,408,410,412..415,420..421,424,427..435,446,448,453,455..488,492,495,507..510,515..517,522..523,533..535,544,548..555,557,559,561,568..570,572,575..576,581..584,599..603,608..613,622..625,627..630,637..640,646..649,658..659,661..662,667..668,670,672..673,675..676,679..681,715,720..721,724,726,729,732,736} (233 alike) : DataTypeConversion  OutDataTypeStr=uint8
  UnitConverter{5,7,29..40,43,46,48,50,52,54..62,64,66,68,70..78,80,82,84,86,88,90,92,94,96..102,104,106,108,110,112..126,128..132,134,136,138,140,142..146,148,150..156,163..164,168..178,181,183..184,186..200,202..210,212,231..233,240..244,246..248,250..251,257,260,318,393..394,400..401,403,406..407,409,411,416..417,419,422..423,425..426,436..438,442..443,445,447,449..452,454,489..490,494,497..499,502..503,518..521,524,536..543,545,547,556,558,560,562..567,571,573..574,577..580,589..598,604..607,614..617,626,631,641..645,660,669,671,674,682..685,694..701,710..714,716,722..723,725,727..728,730,733..735} (276 alike) : DataTypeConversion  OutDataTypeStr=boolean
  UnitConverter{3..4,45,47,49,51,53,93,95,103,105,107,109,111,157,162,185,395..397,418,439..441,444,491,504..506,511..514,525..532,546,585..588,633..636,677..678,686..693,702..709,717..719,731} (72 alike) : DataTypeConversion  OutDataTypeStr=single
  UnitConverter{17..20,496,500..501} (7 alike) : DataTypeConversion  OutDataTypeStr=uint16
  UnitConverter{262..307,309..317,319..392,398,493,618..621,632,650..657,663..666} (148 alike) : DataTypeConversion  OutDataTypeStr=uint32
  VACC_HVTHCMSysAvail_enum_Inproc : FVT_lib/outp/OverrideAndLimit  SystemSampleTime=-1  VariantActivationTime=update diagram  Latency=0  AutoFrameSizeCalculation=off
      link override Signal_Limit/_maxval: Value=KOUTP_HVTHCMSysAvail_enum_maxval
      link override Signal_Limit/_minval: Value=KOUTP_HVTHCMSysAvail_enum_minval
      link override Signal_Override/_ovrdflg: Value=KOUTP_HVTHCMSysAvail_enum_ovrdflg
      link override Signal_Override/_ovrdval: Value=KOUTP_HVTHCMSysAvail_enum_ovrdval
  VACC_LVBattVoltSta_enum_Inproc : FVT_lib/outp/OverrideAndLimit  SystemSampleTime=-1  VariantActivationTime=update diagram  Latency=0  AutoFrameSizeCalculation=off
      link override Signal_Limit/_maxval: Value=KOUTP_LVBattVoltSta_enum_maxval
      link override Signal_Limit/_minval: Value=KOUTP_LVBattVoltSta_enum_minval
      link override Signal_Override/_ovrdflg: Value=KOUTP_LVBattVoltSta_enum_ovrdflg
      link override Signal_Override/_ovrdval: Value=KOUTP_LVBattVoltSta_enum_ovrdval
  VACC_VehHVPwrAvail4THCM_W_Inproc : FVT_lib/outp/OverrideAndLimit  SystemSampleTime=-1  VariantActivationTime=update diagram  Latency=0  AutoFrameSizeCalculation=off
      link override Signal_Limit/_maxval: Value=KOUTP_VehHVPwrAvail4THCM_W_maxval
      link override Signal_Limit/_minval: Value=KOUTP_VehHVPwrAvail4THCM_W_minval
      link override Signal_Override/_ovrdflg: Value=KOUTP_VehHVPwrAvail4THCM_W_ovrdflg
      link override Signal_Override/_ovrdval: Value=KOUTP_VehHVPwrAvail4THCM_W_ovrdval
  VAPM_ABSActiveTimeOut_flg_Inproc : FVT_lib/outp/OverrideAndLimit  SystemSampleTime=-1  VariantActivationTime=update diagram  Latency=0  AutoFrameSizeCalculation=off
      link override Signal_Limit/_maxval: Value=KOUTP_ABSActiveTimeOut_flg_maxval
      link override Signal_Limit/_minval: Value=KOUTP_ABSActiveTimeOut_flg_minval
      link override Signal_Override/_ovrdflg: Value=KOUTP_ABSActiveTimeOut_flg_ovrdflg
      link override Signal_Override/_ovrdval: Value=KOUTP_ABSActiveTimeOut_flg_ovrdval
  VAPM_ABSActive_flg_Inproc : FVT_lib/outp/OverrideAndLimit  SystemSampleTime=-1  VariantActivationTime=update diagram  Latency=0  AutoFrameSizeCalculation=off
      link override Signal_Limit/_maxval: Value=KOUTP_ABSActive_flg_maxval
      link override Signal_Limit/_minval: Value=KOUTP_ABSActive_flg_minval
      link override Signal_Override/_ovrdflg: Value=KOUTP_ABSActive_flg_ovrdflg
      link override Signal_Override/_ovrdval: Value=KOUTP_ABSActive_flg_ovrdval
  VAPM_APSAngleTarget_Deg_Inproc : FVT_lib/outp/OverrideAndLimit  SystemSampleTime=-1  VariantActivationTime=update diagram  Latency=0  AutoFrameSizeCalculation=off
      link override Signal_Limit/_maxval: Value=KOUTP_APSAngleTarget_Deg_maxval
      link override Signal_Limit/_minval: Value=KOUTP_APSAngleTarget_Deg_minval
      link override Signal_Override/_ovrdflg: Value=KOUTP_APSAngleTarget_Deg_ovrdflg
      link override Signal_Override/_ovrdval: Value=KOUTP_APSAngleTarget_Deg_ovrdval
  VAPM_APSDFLL_cm_Inproc : FVT_lib/outp/OverrideAndLimit  SystemSampleTime=-1  VariantActivationTime=update diagram  Latency=0  AutoFrameSizeCalculation=off
      link override Signal_Limit/_maxval: Value=KOUTP_APSDFLL_cm_maxval
      link override Signal_Limit/_minval: Value=KOUTP_APSDFLL_cm_minval
      link override Signal_Override/_ovrdflg: Value=KOUTP_APSDFLL_cm_ovrdflg
      link override Signal_Override/_ovrdval: Value=KOUTP_APSDFLL_cm_ovrdval
  VAPM_APSDFLR_cm_Inproc : FVT_lib/outp/OverrideAndLimit  SystemSampleTime=-1  VariantActivationTime=update diagram  Latency=0  AutoFrameSizeCalculation=off
      link override Signal_Limit/_maxval: Value=KOUTP_APSDFLR_cm_maxval
      link override Signal_Limit/_minval: Value=KOUTP_APSDFLR_cm_minval
      link override Signal_Override/_ovrdflg: Value=KOUTP_APSDFLR_cm_ovrdflg
      link override Signal_Override/_ovrdval: Value=KOUTP_APSDFLR_cm_ovrdval
  VAPM_APSDRLL_cm_Inproc : FVT_lib/outp/OverrideAndLimit  SystemSampleTime=-1  VariantActivationTime=update diagram  Latency=0  AutoFrameSizeCalculation=off
      link override Signal_Limit/_maxval: Value=KOUTP_APSDRLL_cm_maxval
      link override Signal_Limit/_minval: Value=KOUTP_APSDRLL_cm_minval
      link override Signal_Override/_ovrdflg: Value=KOUTP_APSDRLL_cm_ovrdflg
      link override Signal_Override/_ovrdval: Value=KOUTP_APSDRLL_cm_ovrdval
  VAPM_APSDRLR_cm_Inproc : FVT_lib/outp/OverrideAndLimit  SystemSampleTime=-1  VariantActivationTime=update diagram  Latency=0  AutoFrameSizeCalculation=off
      link override Signal_Limit/_maxval: Value=KOUTP_APSDRLR_cm_maxval
      link override Signal_Limit/_minval: Value=KOUTP_APSDRLR_cm_minval
      link override Signal_Override/_ovrdflg: Value=KOUTP_APSDRLR_cm_ovrdflg
      link override Signal_Override/_ovrdval: Value=KOUTP_APSDRLR_cm_ovrdval
  VAPM_APSExitCondition_enum_Inproc : FVT_lib/outp/OverrideAndLimit  SystemSampleTime=-1  VariantActivationTime=update diagram  Latency=0  AutoFrameSizeCalculation=off
      link override Signal_Limit/_maxval: Value=KOUTP_APSExitCondition_enum_maxval
      link override Signal_Limit/_minval: Value=KOUTP_APSExitCondition_enum_minval
      link override Signal_Override/_ovrdflg: Value=KOUTP_APSExitCondition_enum_ovrdflg
      link override Signal_Override/_ovrdval: Value=KOUTP_APSExitCondition_enum_ovrdval
  VAPM_APSHWVer_enum_Inproc : FVT_lib/outp/OverrideAndLimit  SystemSampleTime=-1  VariantActivationTime=update diagram  Latency=0  AutoFrameSizeCalculation=off
      link override Signal_Limit/_maxval: Value=KOUTP_APSHWVer_enum_maxval
      link override Signal_Limit/_minval: Value=KOUTP_APSHWVer_enum_minval
      link override Signal_Override/_ovrdflg: Value=KOUTP_APSHWVer_enum_ovrdflg
      link override Signal_Override/_ovrdval: Value=KOUTP_APSHWVer_enum_ovrdval
  VAPM_APSProgressPCT_pct_Inproc : FVT_lib/outp/OverrideAndLimit  SystemSampleTime=-1  VariantActivationTime=update diagram  Latency=0  AutoFrameSizeCalculation=off
      link override Signal_Limit/_maxval: Value=KOUTP_APSProgressPCT_pct_maxval
      link override Signal_Limit/_minval: Value=KOUTP_APSProgressPCT_pct_minval
      link override Signal_Override/_ovrdflg: Value=KOUTP_APSProgressPCT_pct_ovrdflg
      link override Signal_Override/_ovrdval: Value=KOUTP_APSProgressPCT_pct_ovrdval
  VAPM_APSRQDisplay_enum_Inproc : FVT_lib/outp/OverrideAndLimit  SystemSampleTime=-1  VariantActivationTime=update diagram  Latency=0  AutoFrameSizeCalculation=off
      link override Signal_Limit/_maxval: Value=KOUTP_APSRQDisplay_enum_maxval
      link override Signal_Limit/_minval: Value=KOUTP_APSRQDisplay_enum_minval
      link override Signal_Override/_ovrdflg: Value=KOUTP_APSRQDisplay_enum_ovrdflg
      link override Signal_Override/_ovrdval: Value=KOUTP_APSRQDisplay_enum_ovrdval
  VAPM_APSRqEPASCtrl_flg_Inproc : FVT_lib/outp/OverrideAndLimit  SystemSampleTime=-1  VariantActivationTime=update diagram  Latency=0  AutoFrameSizeCalculation=off
      link override Signal_Limit/_maxval: Value=KOUTP_APSRqEPASCtrl_flg_maxval
      link override Signal_Limit/_minval: Value=KOUTP_APSRqEPASCtrl_flg_minval
      link override Signal_Override/_ovrdflg: Value=KOUTP_APSRqEPASCtrl_flg_ovrdflg
      link override Signal_Override/_ovrdval: Value=KOUTP_APSRqEPASCtrl_flg_ovrdval
  VAPM_APSSWVer_enum_Inproc : FVT_lib/outp/OverrideAndLimit  SystemSampleTime=-1  VariantActivationTime=update diagram  Latency=0  AutoFrameSizeCalculation=off
      link override Signal_Limit/_maxval: Value=KOUTP_APSSWVer_enum_maxval
      link override Signal_Limit/_minval: Value=KOUTP_APSSWVer_enum_minval
      link override Signal_Override/_ovrdflg: Value=KOUTP_APSSWVer_enum_ovrdflg
      link override Signal_Override/_ovrdval: Value=KOUTP_APSSWVer_enum_ovrdval
  VAPM_APSVRqEPASCtrl_flg_Inproc : FVT_lib/outp/OverrideAndLimit  SystemSampleTime=-1  VariantActivationTime=update diagram  Latency=0  AutoFrameSizeCalculation=off
      link override Signal_Limit/_maxval: Value=KOUTP_APSVRqEPASCtrl_flg_maxval
      link override Signal_Limit/_minval: Value=KOUTP_APSVRqEPASCtrl_flg_minval
      link override Signal_Override/_ovrdflg: Value=KOUTP_APSVRqEPASCtrl_flg_ovrdflg
      link override Signal_Override/_ovrdval: Value=KOUTP_APSVRqEPASCtrl_flg_ovrdval
  VAPM_AVMErrSTATimeOut_flg_Inproc : FVT_lib/outp/OverrideAndLimit  SystemSampleTime=-1  VariantActivationTime=update diagram  Latency=0  AutoFrameSizeCalculation=off
      link override Signal_Limit/_maxval: Value=KOUTP_AVMErrSTATimeOut_flg_maxval
      link override Signal_Limit/_minval: Value=KOUTP_AVMErrSTATimeOut_flg_minval
      link override Signal_Override/_ovrdflg: Value=KOUTP_AVMErrSTATimeOut_flg_ovrdflg
      link override Signal_Override/_ovrdval: Value=KOUTP_AVMErrSTATimeOut_flg_ovrdval
  VAPM_AVMErrSTA_flg_Inproc : FVT_lib/outp/OverrideAndLimit  SystemSampleTime=-1  VariantActivationTime=update diagram  Latency=0  AutoFrameSizeCalculation=off
      link override Signal_Limit/_maxval: Value=KOUTP_AVMErrSTA_flg_maxval
      link override Signal_Limit/_minval: Value=KOUTP_AVMErrSTA_flg_minval
      link override Signal_Override/_ovrdflg: Value=KOUTP_AVMErrSTA_flg_ovrdflg
      link override Signal_Override/_ovrdval: Value=KOUTP_AVMErrSTA_flg_ovrdval
  VAPM_AVMParkingmodeTimeOut_flg_Inproc : FVT_lib/outp/OverrideAndLimit  SystemSampleTime=-1  VariantActivationTime=update diagram  Latency=0  AutoFrameSizeCalculation=off
      link override Signal_Limit/_maxval: Value=KOUTP_AVMParkingmodeTimeOut_flg_maxval
      link override Signal_Limit/_minval: Value=KOUTP_AVMParkingmodeTimeOut_flg_minval
      link override Signal_Override/_ovrdflg: Value=KOUTP_AVMParkingmodeTimeOut_flg_ovrdflg
      link override Signal_Override/_ovrdval: Value=KOUTP_AVMParkingmodeTimeOut_flg_ovrdval
  VAPM_AVMParkingmode_enum_Inproc : FVT_lib/outp/OverrideAndLimit  SystemSampleTime=-1  VariantActivationTime=update diagram  Latency=0  AutoFrameSizeCalculation=off
      link override Signal_Limit/_maxval: Value=KOUTP_AVMParkingmode_enum_maxval
      link override Signal_Limit/_minval: Value=KOUTP_AVMParkingmode_enum_minval
      link override Signal_Override/_ovrdflg: Value=KOUTP_AVMParkingmode_enum_ovrdflg
      link override Signal_Override/_ovrdval: Value=KOUTP_AVMParkingmode_enum_ovrdval
  VAPM_AVMparkingcancelTimeOut_flg_Inproc : FVT_lib/outp/OverrideAndLimit  SystemSampleTime=-1  VariantActivationTime=update diagram  Latency=0  AutoFrameSizeCalculation=off
      link override Signal_Limit/_maxval: Value=KOUTP_AVMparkingcancelTimeOut_flg_maxval
      link override Signal_Limit/_minval: Value=KOUTP_AVMparkingcancelTimeOut_flg_minval
      link override Signal_Override/_ovrdflg: Value=KOUTP_AVMparkingcancelTimeOut_flg_ovrdflg
      link override Signal_Override/_ovrdval: Value=KOUTP_AVMparkingcancelTimeOut_flg_ovrdval
  VAPM_AVMparkingcancel_enum_Inproc : FVT_lib/outp/OverrideAndLimit  SystemSampleTime=-1  VariantActivationTime=update diagram  Latency=0  AutoFrameSizeCalculation=off
      link override Signal_Limit/_maxval: Value=KOUTP_AVMparkingcancel_enum_maxval
      link override Signal_Limit/_minval: Value=KOUTP_AVMparkingcancel_enum_minval
      link override Signal_Override/_ovrdflg: Value=KOUTP_AVMparkingcancel_enum_ovrdflg
      link override Signal_Override/_ovrdval: Value=KOUTP_AVMparkingcancel_enum_ovrdval
  VAPM_AVMparkingexcuteTimeOut_flg_Inproc : FVT_lib/outp/OverrideAndLimit  SystemSampleTime=-1  VariantActivationTime=update diagram  Latency=0  AutoFrameSizeCalculation=off
      link override Signal_Limit/_maxval: Value=KOUTP_AVMparkingexcuteTimeOut_flg_maxval
      link override Signal_Limit/_minval: Value=KOUTP_AVMparkingexcuteTimeOut_flg_minval
      link override Signal_Override/_ovrdflg: Value=KOUTP_AVMparkingexcuteTimeOut_flg_ovrdflg
      link override Signal_Override/_ovrdval: Value=KOUTP_AVMparkingexcuteTimeOut_flg_ovrdval
  VAPM_AVMparkingexcute_enum_Inproc : FVT_lib/outp/OverrideAndLimit  SystemSampleTime=-1  VariantActivationTime=update diagram  Latency=0  AutoFrameSizeCalculation=off
      link override Signal_Limit/_maxval: Value=KOUTP_AVMparkingexcute_enum_maxval
      link override Signal_Limit/_minval: Value=KOUTP_AVMparkingexcute_enum_minval
      link override Signal_Override/_ovrdflg: Value=KOUTP_AVMparkingexcute_enum_ovrdflg
      link override Signal_Override/_ovrdval: Value=KOUTP_AVMparkingexcute_enum_ovrdval
  VAPM_BrkPedalPosTimeOut_flg_Inproc : FVT_lib/outp/OverrideAndLimit  SystemSampleTime=-1  VariantActivationTime=update diagram  Latency=0  AutoFrameSizeCalculation=off
      link override Signal_Limit/_maxval: Value=KOUTP_BrkPedalPosTimeOut_flg_maxval
      link override Signal_Limit/_minval: Value=KOUTP_BrkPedalPosTimeOut_flg_minval
      link override Signal_Override/_ovrdflg: Value=KOUTP_BrkPedalPosTimeOut_flg_ovrdflg
      link override Signal_Override/_ovrdval: Value=KOUTP_BrkPedalPosTimeOut_flg_ovrdval
  VAPM_BrkPedalPos_pct_Inproc : FVT_lib/outp/OverrideAndLimit  SystemSampleTime=-1  VariantActivationTime=update diagram  Latency=0  AutoFrameSizeCalculation=off
      link override Signal_Limit/_maxval: Value=KOUTP_BrkPedalPos_pct_maxval
      link override Signal_Limit/_minval: Value=KOUTP_BrkPedalPos_pct_minval
      link override Signal_Override/_ovrdflg: Value=KOUTP_BrkPedalPos_pct_ovrdflg
      link override Signal_Override/_ovrdval: Value=KOUTP_BrkPedalPos_pct_ovrdval
  VAPM_BrkSwStaTimeOut_flg_Inproc : FVT_lib/outp/OverrideAndLimit  SystemSampleTime=-1  VariantActivationTime=update diagram  Latency=0  AutoFrameSizeCalculation=off
      link override Signal_Limit/_maxval: Value=KOUTP_BrkSwStaTimeOut_flg_maxval
      link override Signal_Limit/_minval: Value=KOUTP_BrkSwStaTimeOut_flg_minval
      link override Signal_Override/_ovrdflg: Value=KOUTP_BrkSwStaTimeOut_flg_ovrdflg
      link override Signal_Override/_ovrdval: Value=KOUTP_BrkSwStaTimeOut_flg_ovrdval
  VAPM_BrkSwSta_flg_Inproc : FVT_lib/outp/OverrideAndLimit  SystemSampleTime=-1  VariantActivationTime=update diagram  Latency=0  AutoFrameSizeCalculation=off
      link override Signal_Limit/_maxval: Value=KOUTP_BrkSwSta_flg_maxval
      link override Signal_Limit/_minval: Value=KOUTP_BrkSwSta_flg_minval
      link override Signal_Override/_ovrdflg: Value=KOUTP_BrkSwSta_flg_ovrdflg
      link override Signal_Override/_ovrdval: Value=KOUTP_BrkSwSta_flg_ovrdval
  VAPM_BrkSwVTimeOut_flg_Inproc : FVT_lib/outp/OverrideAndLimit  SystemSampleTime=-1  VariantActivationTime=update diagram  Latency=0  AutoFrameSizeCalculation=off
      link override Signal_Limit/_maxval: Value=KOUTP_BrkSwVTimeOut_flg_maxval
      link override Signal_Limit/_minval: Value=KOUTP_BrkSwVTimeOut_flg_minval
      link override Signal_Override/_ovrdflg: Value=KOUTP_BrkSwVTimeOut_flg_ovrdflg
      link override Signal_Override/_ovrdval: Value=KOUTP_BrkSwVTimeOut_flg_ovrdval
  VAPM_BrkSwV_flg_Inproc : FVT_lib/outp/OverrideAndLimit  SystemSampleTime=-1  VariantActivationTime=update diagram  Latency=0  AutoFrameSizeCalculation=off
      link override Signal_Limit/_maxval: Value=KOUTP_BrkSwV_flg_maxval
      link override Signal_Limit/_minval: Value=KOUTP_BrkSwV_flg_minval
      link override Signal_Override/_ovrdflg: Value=KOUTP_BrkSwV_flg_ovrdflg
      link override Signal_Override/_ovrdval: Value=KOUTP_BrkSwV_flg_ovrdval
  VAPM_CAASSta_enum_Inproc : FVT_lib/outp/OverrideAndLimit  SystemSampleTime=-1  VariantActivationTime=update diagram  Latency=0  AutoFrameSizeCalculation=off
      link override Signal_Limit/_maxval: Value=KOUTP_CAASSta_enum_maxval
      link override Signal_Limit/_minval: Value=KOUTP_CAASSta_enum_minval
      link override Signal_Override/_ovrdflg: Value=KOUTP_CAASSta_enum_ovrdflg
      link override Signal_Override/_ovrdval: Value=KOUTP_CAASSta_enum_ovrdval
  VAPM_CAASSwTimeOut_flg_Inproc : FVT_lib/outp/OverrideAndLimit  SystemSampleTime=-1  VariantActivationTime=update diagram  Latency=0  AutoFrameSizeCalculation=off
      link override Signal_Limit/_maxval: Value=KOUTP_CAASSwTimeOut_flg_maxval
      link override Signal_Limit/_minval: Value=KOUTP_CAASSwTimeOut_flg_minval
      link override Signal_Override/_ovrdflg: Value=KOUTP_CAASSwTimeOut_flg_ovrdflg
      link override Signal_Override/_ovrdval: Value=KOUTP_CAASSwTimeOut_flg_ovrdval
  VAPM_CAASSw_enum_Inproc : FVT_lib/outp/OverrideAndLimit  SystemSampleTime=-1  VariantActivationTime=update diagram  Latency=0  AutoFrameSizeCalculation=off
      link override Signal_Limit/_maxval: Value=KOUTP_CAASSw_enum_maxval
      link override Signal_Limit/_minval: Value=KOUTP_CAASSw_enum_minval
      link override Signal_Override/_ovrdflg: Value=KOUTP_CAASSw_enum_ovrdflg
      link override Signal_Override/_ovrdval: Value=KOUTP_CAASSw_enum_ovrdval
  VAPM_Chime_enum_Inproc : FVT_lib/outp/OverrideAndLimit  SystemSampleTime=-1  VariantActivationTime=update diagram  Latency=0  AutoFrameSizeCalculation=off
      link override Signal_Limit/_maxval: Value=KOUTP_Chime_enum_maxval
      link override Signal_Limit/_minval: Value=KOUTP_Chime_enum_minval
      link override Signal_Override/_ovrdflg: Value=KOUTP_Chime_enum_ovrdflg
      link override Signal_Override/_ovrdval: Value=KOUTP_Chime_enum_ovrdval
  VAPM_ChrgPlugSta_enum_Inproc : FVT_lib/outp/OverrideAndLimit  SystemSampleTime=-1  VariantActivationTime=update diagram  Latency=0  AutoFrameSizeCalculation=off
      link override Signal_Limit/_maxval: Value=KOUTP_ChrgPlugSta_enum_maxval
      link override Signal_Limit/_minval: Value=KOUTP_ChrgPlugSta_enum_minval
      link override Signal_Override/_ovrdflg: Value=KOUTP_ChrgPlugSta_enum_ovrdflg
      link override Signal_Override/_ovrdval: Value=KOUTP_ChrgPlugSta_enum_ovrdval
  VAPM_DriIntendTimeOut_flg_Inproc : FVT_lib/outp/OverrideAndLimit  SystemSampleTime=-1  VariantActivationTime=update diagram  Latency=0  AutoFrameSizeCalculation=off
      link override Signal_Limit/_maxval: Value=KOUTP_DriIntendTimeOut_flg_maxval
      link override Signal_Limit/_minval: Value=KOUTP_DriIntendTimeOut_flg_minval
      link override Signal_Override/_ovrdflg: Value=KOUTP_DriIntendTimeOut_flg_ovrdflg
      link override Signal_Override/_ovrdval: Value=KOUTP_DriIntendTimeOut_flg_ovrdval
  VAPM_DriIntend_enum_Inproc : FVT_lib/outp/OverrideAndLimit  SystemSampleTime=-1  VariantActivationTime=update diagram  Latency=0  AutoFrameSizeCalculation=off
      link override Signal_Limit/_maxval: Value=KOUTP_DriIntend_enum_maxval
      link override Signal_Limit/_minval: Value=KOUTP_DriIntend_enum_minval
      link override Signal_Override/_ovrdflg: Value=KOUTP_DriIntend_enum_ovrdflg
      link override Signal_Override/_ovrdval: Value=KOUTP_DriIntend_enum_ovrdval
  VAPM_DriverSeatBeltCmdTimeOut_flg_Inproc : FVT_lib/outp/OverrideAndLimit  SystemSampleTime=-1  VariantActivationTime=update diagram  Latency=0  AutoFrameSizeCalculation=off
      link override Signal_Limit/_maxval: Value=KOUTP_DriverSeatBeltCmdTimeOut_flg_maxval
      link override Signal_Limit/_minval: Value=KOUTP_DriverSeatBeltCmdTimeOut_flg_minval
      link override Signal_Override/_ovrdflg: Value=KOUTP_DriverSeatBeltCmdTimeOut_flg_ovrdflg
      link override Signal_Override/_ovrdval: Value=KOUTP_DriverSeatBeltCmdTimeOut_flg_ovrdval
  VAPM_DriverSeatBeltCmd_flg_Inproc : FVT_lib/outp/OverrideAndLimit  SystemSampleTime=-1  VariantActivationTime=update diagram  Latency=0  AutoFrameSizeCalculation=off
      link override Signal_Limit/_maxval: Value=KOUTP_DriverSeatBeltCmd_flg_maxval
      link override Signal_Limit/_minval: Value=KOUTP_DriverSeatBeltCmd_flg_minval
      link override Signal_Override/_ovrdflg: Value=KOUTP_DriverSeatBeltCmd_flg_ovrdflg
      link override Signal_Override/_ovrdval: Value=KOUTP_DriverSeatBeltCmd_flg_ovrdval
  VAPM_EPBErrStaTimeOut_flg_Inproc : FVT_lib/outp/OverrideAndLimit  SystemSampleTime=-1  VariantActivationTime=update diagram  Latency=0  AutoFrameSizeCalculation=off
      link override Signal_Limit/_maxval: Value=KOUTP_EPBErrStaTimeOut_flg_maxval
      link override Signal_Limit/_minval: Value=KOUTP_EPBErrStaTimeOut_flg_minval
      link override Signal_Override/_ovrdflg: Value=KOUTP_EPBErrStaTimeOut_flg_ovrdflg
      link override Signal_Override/_ovrdval: Value=KOUTP_EPBErrStaTimeOut_flg_ovrdval
  VAPM_EPBErrSta_enum_Inproc : FVT_lib/outp/OverrideAndLimit  SystemSampleTime=-1  VariantActivationTime=update diagram  Latency=0  AutoFrameSizeCalculation=off
      link override Signal_Limit/_maxval: Value=KOUTP_EPBErrSta_enum_maxval
      link override Signal_Limit/_minval: Value=KOUTP_EPBErrSta_enum_minval
      link override Signal_Override/_ovrdflg: Value=KOUTP_EPBErrSta_enum_ovrdflg
      link override Signal_Override/_ovrdval: Value=KOUTP_EPBErrSta_enum_ovrdval
  VAPM_EPBExtApplyAvailTimeOut_flg_Inproc : FVT_lib/outp/OverrideAndLimit  SystemSampleTime=-1  VariantActivationTime=update diagram  Latency=0  AutoFrameSizeCalculation=off
      link override Signal_Limit/_maxval: Value=KOUTP_EPBExtApplyAvailTimeOut_flg_maxval
      link override Signal_Limit/_minval: Value=KOUTP_EPBExtApplyAvailTimeOut_flg_minval
      link override Signal_Override/_ovrdflg: Value=KOUTP_EPBExtApplyAvailTimeOut_flg_ovrdflg
      link override Signal_Override/_ovrdval: Value=KOUTP_EPBExtApplyAvailTimeOut_flg_ovrdval
  VAPM_EPBExtApplyAvail_flg_Inproc : FVT_lib/outp/OverrideAndLimit  SystemSampleTime=-1  VariantActivationTime=update diagram  Latency=0  AutoFrameSizeCalculation=off
      link override Signal_Limit/_maxval: Value=KOUTP_EPBExtApplyAvail_flg_maxval
      link override Signal_Limit/_minval: Value=KOUTP_EPBExtApplyAvail_flg_minval
      link override Signal_Override/_ovrdflg: Value=KOUTP_EPBExtApplyAvail_flg_ovrdflg
      link override Signal_Override/_ovrdval: Value=KOUTP_EPBExtApplyAvail_flg_ovrdval
  VAPM_EPBExtReleaseAvailTimeOut_flg_Inproc : FVT_lib/outp/OverrideAndLimit  SystemSampleTime=-1  VariantActivationTime=update diagram  Latency=0  AutoFrameSizeCalculation=off
      link override Signal_Limit/_maxval: Value=KOUTP_EPBExtReleaseAvailTimeOut_flg_maxval
      link override Signal_Limit/_minval: Value=KOUTP_EPBExtReleaseAvailTimeOut_flg_minval
      link override Signal_Override/_ovrdflg: Value=KOUTP_EPBExtReleaseAvailTimeOut_flg_ovrdflg
      link override Signal_Override/_ovrdval: Value=KOUTP_EPBExtReleaseAvailTimeOut_flg_ovrdval
  VAPM_EPBExtReleaseAvail_flg_Inproc : FVT_lib/outp/OverrideAndLimit  SystemSampleTime=-1  VariantActivationTime=update diagram  Latency=0  AutoFrameSizeCalculation=off
      link override Signal_Limit/_maxval: Value=KOUTP_EPBExtReleaseAvail_flg_maxval
      link override Signal_Limit/_minval: Value=KOUTP_EPBExtReleaseAvail_flg_minval
      link override Signal_Override/_ovrdflg: Value=KOUTP_EPBExtReleaseAvail_flg_ovrdflg
      link override Signal_Override/_ovrdval: Value=KOUTP_EPBExtReleaseAvail_flg_ovrdval
  VAPM_EPBStaTimeOut_flg_Inproc : FVT_lib/outp/OverrideAndLimit  SystemSampleTime=-1  VariantActivationTime=update diagram  Latency=0  AutoFrameSizeCalculation=off
      link override Signal_Limit/_maxval: Value=KOUTP_EPBStaTimeOut_flg_maxval
      link override Signal_Limit/_minval: Value=KOUTP_EPBStaTimeOut_flg_minval
      link override Signal_Override/_ovrdflg: Value=KOUTP_EPBStaTimeOut_flg_ovrdflg
      link override Signal_Override/_ovrdval: Value=KOUTP_EPBStaTimeOut_flg_ovrdval
  VAPM_EPBSta_enum_Inproc : FVT_lib/outp/OverrideAndLimit  SystemSampleTime=-1  VariantActivationTime=update diagram  Latency=0  AutoFrameSizeCalculation=off
      link override Signal_Limit/_maxval: Value=KOUTP_EPBSta_enum_maxval
      link override Signal_Limit/_minval: Value=KOUTP_EPBSta_enum_minval
      link override Signal_Override/_ovrdflg: Value=KOUTP_EPBSta_enum_ovrdflg
      link override Signal_Override/_ovrdval: Value=KOUTP_EPBSta_enum_ovrdval
  VAPM_EPSAOIControlTimeOut_flg_Inproc : FVT_lib/outp/OverrideAndLimit  SystemSampleTime=-1  VariantActivationTime=update diagram  Latency=0  AutoFrameSizeCalculation=off
      link override Signal_Limit/_maxval: Value=KOUTP_EPSAOIControlTimeOut_flg_maxval
      link override Signal_Limit/_minval: Value=KOUTP_EPSAOIControlTimeOut_flg_minval
      link override Signal_Override/_ovrdflg: Value=KOUTP_EPSAOIControlTimeOut_flg_ovrdflg
      link override Signal_Override/_ovrdval: Value=KOUTP_EPSAOIControlTimeOut_flg_ovrdval
  VAPM_EPSAOIControl_enum_Inproc : FVT_lib/outp/OverrideAndLimit  SystemSampleTime=-1  VariantActivationTime=update diagram  Latency=0  AutoFrameSizeCalculation=off
      link override Signal_Limit/_maxval: Value=KOUTP_EPSAOIControl_enum_maxval
      link override Signal_Limit/_minval: Value=KOUTP_EPSAOIControl_enum_minval
      link override Signal_Override/_ovrdflg: Value=KOUTP_EPSAOIControl_enum_ovrdflg
      link override Signal_Override/_ovrdval: Value=KOUTP_EPSAOIControl_enum_ovrdval
  VAPM_ESCAPSStaTimeOut_flg_Inproc : FVT_lib/outp/OverrideAndLimit  SystemSampleTime=-1  VariantActivationTime=update diagram  Latency=0  AutoFrameSizeCalculation=off
      link override Signal_Limit/_maxval: Value=KOUTP_ESCAPSStaTimeOut_flg_maxval
      link override Signal_Limit/_minval: Value=KOUTP_ESCAPSStaTimeOut_flg_minval
      link override Signal_Override/_ovrdflg: Value=KOUTP_ESCAPSStaTimeOut_flg_ovrdflg
      link override Signal_Override/_ovrdval: Value=KOUTP_ESCAPSStaTimeOut_flg_ovrdval
  VAPM_ESCAPSSta_enum_Inproc : FVT_lib/outp/OverrideAndLimit  SystemSampleTime=-1  VariantActivationTime=update diagram  Latency=0  AutoFrameSizeCalculation=off
      link override Signal_Limit/_maxval: Value=KOUTP_ESCAPSSta_enum_maxval
      link override Signal_Limit/_minval: Value=KOUTP_ESCAPSSta_enum_minval
      link override Signal_Override/_ovrdflg: Value=KOUTP_ESCAPSSta_enum_ovrdflg
      link override Signal_Override/_ovrdval: Value=KOUTP_ESCAPSSta_enum_ovrdval
  VAPM_ESCStandstillTimeOut_flg_Inproc : FVT_lib/outp/OverrideAndLimit  SystemSampleTime=-1  VariantActivationTime=update diagram  Latency=0  AutoFrameSizeCalculation=off
      link override Signal_Limit/_maxval: Value=KOUTP_ESCStandstillTimeOut_flg_maxval
      link override Signal_Limit/_minval: Value=KOUTP_ESCStandstillTimeOut_flg_minval
      link override Signal_Override/_ovrdflg: Value=KOUTP_ESCStandstillTimeOut_flg_ovrdflg
      link override Signal_Override/_ovrdval: Value=KOUTP_ESCStandstillTimeOut_flg_ovrdval
  VAPM_ESCStandstill_flg_Inproc : FVT_lib/outp/OverrideAndLimit  SystemSampleTime=-1  VariantActivationTime=update diagram  Latency=0  AutoFrameSizeCalculation=off
      link override Signal_Limit/_maxval: Value=KOUTP_ESCStandstill_flg_maxval
      link override Signal_Limit/_minval: Value=KOUTP_ESCStandstill_flg_minval
      link override Signal_Override/_ovrdflg: Value=KOUTP_ESCStandstill_flg_ovrdflg
      link override Signal_Override/_ovrdval: Value=KOUTP_ESCStandstill_flg_ovrdval
  VAPM_FSOffSwTimeOut_flg_Inproc : FVT_lib/outp/OverrideAndLimit  SystemSampleTime=-1  VariantActivationTime=update diagram  Latency=0  AutoFrameSizeCalculation=off
      link override Signal_Limit/_maxval: Value=KOUTP_FSOffSwTimeOut_flg_maxval
      link override Signal_Limit/_minval: Value=KOUTP_FSOffSwTimeOut_flg_minval
      link override Signal_Override/_ovrdflg: Value=KOUTP_FSOffSwTimeOut_flg_ovrdflg
      link override Signal_Override/_ovrdval: Value=KOUTP_FSOffSwTimeOut_flg_ovrdval
  VAPM_FSOffSw_enum_Inproc : FVT_lib/outp/OverrideAndLimit  SystemSampleTime=-1  VariantActivationTime=update diagram  Latency=0  AutoFrameSizeCalculation=off
      link override Signal_Limit/_maxval: Value=KOUTP_FSOffSw_enum_maxval
      link override Signal_Limit/_minval: Value=KOUTP_FSOffSw_enum_minval
      link override Signal_Override/_ovrdflg: Value=KOUTP_FSOffSw_enum_ovrdflg
      link override Signal_Override/_ovrdval: Value=KOUTP_FSOffSw_enum_ovrdval
  VAPM_GRADETimeOut_flg_Inproc : FVT_lib/outp/OverrideAndLimit  SystemSampleTime=-1  VariantActivationTime=update diagram  Latency=0  AutoFrameSizeCalculation=off
      link override Signal_Limit/_maxval: Value=KOUTP_GRADETimeOut_flg_maxval
      link override Signal_Limit/_minval: Value=KOUTP_GRADETimeOut_flg_minval
      link override Signal_Override/_ovrdflg: Value=KOUTP_GRADETimeOut_flg_ovrdflg
      link override Signal_Override/_ovrdval: Value=KOUTP_GRADETimeOut_flg_ovrdval
  VAPM_GRADE_Deg_Inproc : FVT_lib/outp/OverrideAndLimit  SystemSampleTime=-1  VariantActivationTime=update diagram  Latency=0  AutoFrameSizeCalculation=off
      link override Signal_Limit/_maxval: Value=KOUTP_GRADE_Deg_maxval
      link override Signal_Limit/_minval: Value=KOUTP_GRADE_Deg_minval
      link override Signal_Override/_ovrdflg: Value=KOUTP_GRADE_Deg_ovrdflg
      link override Signal_Override/_ovrdval: Value=KOUTP_GRADE_Deg_ovrdval
  VAPM_IVIScreenTimeOut_flg_Inproc : FVT_lib/outp/OverrideAndLimit  SystemSampleTime=-1  VariantActivationTime=update diagram  Latency=0  AutoFrameSizeCalculation=off
      link override Signal_Limit/_maxval: Value=KOUTP_IVIScreenTimeOut_flg_maxval
      link override Signal_Limit/_minval: Value=KOUTP_IVIScreenTimeOut_flg_minval
      link override Signal_Override/_ovrdflg: Value=KOUTP_IVIScreenTimeOut_flg_ovrdflg
      link override Signal_Override/_ovrdval: Value=KOUTP_IVIScreenTimeOut_flg_ovrdval
  VAPM_IVIScreen_enum_Inproc : FVT_lib/outp/OverrideAndLimit  SystemSampleTime=-1  VariantActivationTime=update diagram  Latency=0  AutoFrameSizeCalculation=off
      link override Signal_Limit/_maxval: Value=KOUTP_IVIScreen_enum_maxval
      link override Signal_Limit/_minval: Value=KOUTP_IVIScreen_enum_minval
      link override Signal_Override/_ovrdflg: Value=KOUTP_IVIScreen_enum_ovrdflg
      link override Signal_Override/_ovrdval: Value=KOUTP_IVIScreen_enum_ovrdval
  VAPM_IVIStatusTimeOut_flg_Inproc : FVT_lib/outp/OverrideAndLimit  SystemSampleTime=-1  VariantActivationTime=update diagram  Latency=0  AutoFrameSizeCalculation=off
      link override Signal_Limit/_maxval: Value=KOUTP_IVIStatusTimeOut_flg_maxval
      link override Signal_Limit/_minval: Value=KOUTP_IVIStatusTimeOut_flg_minval
      link override Signal_Override/_ovrdflg: Value=KOUTP_IVIStatusTimeOut_flg_ovrdflg
      link override Signal_Override/_ovrdval: Value=KOUTP_IVIStatusTimeOut_flg_ovrdval
  VAPM_IVIStatus_flg_Inproc : FVT_lib/outp/OverrideAndLimit  SystemSampleTime=-1  VariantActivationTime=update diagram  Latency=0  AutoFrameSizeCalculation=off
      link override Signal_Limit/_maxval: Value=KOUTP_IVIStatus_flg_maxval
      link override Signal_Limit/_minval: Value=KOUTP_IVIStatus_flg_minval
      link override Signal_Override/_ovrdflg: Value=KOUTP_IVIStatus_flg_ovrdflg
      link override Signal_Override/_ovrdval: Value=KOUTP_IVIStatus_flg_ovrdval
  VAPM_LFPulseCountTimeOut_flg_Inproc : FVT_lib/outp/OverrideAndLimit  SystemSampleTime=-1  VariantActivationTime=update diagram  Latency=0  AutoFrameSizeCalculation=off
      link override Signal_Limit/_maxval: Value=KOUTP_LFPulseCountTimeOut_flg_maxval
      link override Signal_Limit/_minval: Value=KOUTP_LFPulseCountTimeOut_flg_minval
      link override Signal_Override/_ovrdflg: Value=KOUTP_LFPulseCountTimeOut_flg_ovrdflg
      link override Signal_Override/_ovrdval: Value=KOUTP_LFPulseCountTimeOut_flg_ovrdval
  VAPM_LFPulseCountVTimeOut_flg_Inproc : FVT_lib/outp/OverrideAndLimit  SystemSampleTime=-1  VariantActivationTime=update diagram  Latency=0  AutoFrameSizeCalculation=off
      link override Signal_Limit/_maxval: Value=KOUTP_LFPulseCountVTimeOut_flg_maxval
      link override Signal_Limit/_minval: Value=KOUTP_LFPulseCountVTimeOut_flg_minval
      link override Signal_Override/_ovrdflg: Value=KOUTP_LFPulseCountVTimeOut_flg_ovrdflg
      link override Signal_Override/_ovrdval: Value=KOUTP_LFPulseCountVTimeOut_flg_ovrdval
  VAPM_LFPulseCountV_flg_Inproc : FVT_lib/outp/OverrideAndLimit  SystemSampleTime=-1  VariantActivationTime=update diagram  Latency=0  AutoFrameSizeCalculation=off
      link override Signal_Limit/_maxval: Value=KOUTP_LFPulseCountV_flg_maxval
      link override Signal_Limit/_minval: Value=KOUTP_LFPulseCountV_flg_minval
      link override Signal_Override/_ovrdflg: Value=KOUTP_LFPulseCountV_flg_ovrdflg
      link override Signal_Override/_ovrdval: Value=KOUTP_LFPulseCountV_flg_ovrdval
  VAPM_LFPulseCount_enum_Inproc : FVT_lib/outp/OverrideAndLimit  SystemSampleTime=-1  VariantActivationTime=update diagram  Latency=0  AutoFrameSizeCalculation=off
      link override Signal_Limit/_maxval: Value=KOUTP_LFPulseCount_enum_maxval
      link override Signal_Limit/_minval: Value=KOUTP_LFPulseCount_enum_minval
      link override Signal_Override/_ovrdflg: Value=KOUTP_LFPulseCount_enum_ovrdflg
      link override Signal_Override/_ovrdval: Value=KOUTP_LFPulseCount_enum_ovrdval
  VAPM_LFRawWhlSpeedTimeOut_flg_Inproc : FVT_lib/outp/OverrideAndLimit  SystemSampleTime=-1  VariantActivationTime=update diagram  Latency=0  AutoFrameSizeCalculation=off
      link override Signal_Limit/_maxval: Value=KOUTP_LFRawWhlSpeedTimeOut_flg_maxval
      link override Signal_Limit/_minval: Value=KOUTP_LFRawWhlSpeedTimeOut_flg_minval
      link override Signal_Override/_ovrdflg: Value=KOUTP_LFRawWhlSpeedTimeOut_flg_ovrdflg
      link override Signal_Override/_ovrdval: Value=KOUTP_LFRawWhlSpeedTimeOut_flg_ovrdval
  VAPM_LFRawWhlSpeedVTimeOut_flg_Inproc : FVT_lib/outp/OverrideAndLimit  SystemSampleTime=-1  VariantActivationTime=update diagram  Latency=0  AutoFrameSizeCalculation=off
      link override Signal_Limit/_maxval: Value=KOUTP_LFRawWhlSpeedVTimeOut_flg_maxval
      link override Signal_Limit/_minval: Value=KOUTP_LFRawWhlSpeedVTimeOut_flg_minval
      link override Signal_Override/_ovrdflg: Value=KOUTP_LFRawWhlSpeedVTimeOut_flg_ovrdflg
      link override Signal_Override/_ovrdval: Value=KOUTP_LFRawWhlSpeedVTimeOut_flg_ovrdval
  VAPM_LFRawWhlSpeedV_flg_Inproc : FVT_lib/outp/OverrideAndLimit  SystemSampleTime=-1  VariantActivationTime=update diagram  Latency=0  AutoFrameSizeCalculation=off
      link override Signal_Limit/_maxval: Value=KOUTP_LFRawWhlSpeedV_flg_maxval
      link override Signal_Limit/_minval: Value=KOUTP_LFRawWhlSpeedV_flg_minval
      link override Signal_Override/_ovrdflg: Value=KOUTP_LFRawWhlSpeedV_flg_ovrdflg
      link override Signal_Override/_ovrdval: Value=KOUTP_LFRawWhlSpeedV_flg_ovrdval
  VAPM_LFRawWhlSpeed_kph_Inproc : FVT_lib/outp/OverrideAndLimit  SystemSampleTime=-1  VariantActivationTime=update diagram  Latency=0  AutoFrameSizeCalculation=off
      link override Signal_Limit/_maxval: Value=KOUTP_LFRawWhlSpeed_kph_maxval
      link override Signal_Limit/_minval: Value=KOUTP_LFRawWhlSpeed_kph_minval
      link override Signal_Override/_ovrdflg: Value=KOUTP_LFRawWhlSpeed_kph_ovrdflg
      link override Signal_Override/_ovrdval: Value=KOUTP_LFRawWhlSpeed_kph_ovrdval
  VAPM_LFWhlRotDirTimeOut_flg_Inproc : FVT_lib/outp/OverrideAndLimit  SystemSampleTime=-1  VariantActivationTime=update diagram  Latency=0  AutoFrameSizeCalculation=off
      link override Signal_Limit/_maxval: Value=KOUTP_LFWhlRotDirTimeOut_flg_maxval
      link override Signal_Limit/_minval: Value=KOUTP_LFWhlRotDirTimeOut_flg_minval
      link override Signal_Override/_ovrdflg: Value=KOUTP_LFWhlRotDirTimeOut_flg_ovrdflg
      link override Signal_Override/_ovrdval: Value=KOUTP_LFWhlRotDirTimeOut_flg_ovrdval
  VAPM_LFWhlRotDir_enum_Inproc : FVT_lib/outp/OverrideAndLimit  SystemSampleTime=-1  VariantActivationTime=update diagram  Latency=0  AutoFrameSizeCalculation=off
      link override Signal_Limit/_maxval: Value=KOUTP_LFWhlRotDir_enum_maxval
      link override Signal_Limit/_minval: Value=KOUTP_LFWhlRotDir_enum_minval
      link override Signal_Override/_ovrdflg: Value=KOUTP_LFWhlRotDir_enum_ovrdflg
      link override Signal_Override/_ovrdval: Value=KOUTP_LFWhlRotDir_enum_ovrdval
  VAPM_LRPulseCountTimeOut_flg_Inproc : FVT_lib/outp/OverrideAndLimit  SystemSampleTime=-1  VariantActivationTime=update diagram  Latency=0  AutoFrameSizeCalculation=off
      link override Signal_Limit/_maxval: Value=KOUTP_LRPulseCountTimeOut_flg_maxval
      link override Signal_Limit/_minval: Value=KOUTP_LRPulseCountTimeOut_flg_minval
      link override Signal_Override/_ovrdflg: Value=KOUTP_LRPulseCountTimeOut_flg_ovrdflg
      link override Signal_Override/_ovrdval: Value=KOUTP_LRPulseCountTimeOut_flg_ovrdval
  VAPM_LRPulseCountVTimeOut_flg_Inproc : FVT_lib/outp/OverrideAndLimit  SystemSampleTime=-1  VariantActivationTime=update diagram  Latency=0  AutoFrameSizeCalculation=off
      link override Signal_Limit/_maxval: Value=KOUTP_LRPulseCountVTimeOut_flg_maxval
      link override Signal_Limit/_minval: Value=KOUTP_LRPulseCountVTimeOut_flg_minval
      link override Signal_Override/_ovrdflg: Value=KOUTP_LRPulseCountVTimeOut_flg_ovrdflg
      link override Signal_Override/_ovrdval: Value=KOUTP_LRPulseCountVTimeOut_flg_ovrdval
  VAPM_LRPulseCountV_flg_Inproc : FVT_lib/outp/OverrideAndLimit  SystemSampleTime=-1  VariantActivationTime=update diagram  Latency=0  AutoFrameSizeCalculation=off
      link override Signal_Limit/_maxval: Value=KOUTP_LRPulseCountV_flg_maxval
      link override Signal_Limit/_minval: Value=KOUTP_LRPulseCountV_flg_minval
      link override Signal_Override/_ovrdflg: Value=KOUTP_LRPulseCountV_flg_ovrdflg
      link override Signal_Override/_ovrdval: Value=KOUTP_LRPulseCountV_flg_ovrdval
  VAPM_LRPulseCount_enum_Inproc : FVT_lib/outp/OverrideAndLimit  SystemSampleTime=-1  VariantActivationTime=update diagram  Latency=0  AutoFrameSizeCalculation=off
      link override Signal_Limit/_maxval: Value=KOUTP_LRPulseCount_enum_maxval
      link override Signal_Limit/_minval: Value=KOUTP_LRPulseCount_enum_minval
      link override Signal_Override/_ovrdflg: Value=KOUTP_LRPulseCount_enum_ovrdflg
      link override Signal_Override/_ovrdval: Value=KOUTP_LRPulseCount_enum_ovrdval
  VAPM_LRRawWhlSpeedTimeOut_flg_Inproc : FVT_lib/outp/OverrideAndLimit  SystemSampleTime=-1  VariantActivationTime=update diagram  Latency=0  AutoFrameSizeCalculation=off
      link override Signal_Limit/_maxval: Value=KOUTP_LRRawWhlSpeedTimeOut_flg_maxval
      link override Signal_Limit/_minval: Value=KOUTP_LRRawWhlSpeedTimeOut_flg_minval
      link override Signal_Override/_ovrdflg: Value=KOUTP_LRRawWhlSpeedTimeOut_flg_ovrdflg
      link override Signal_Override/_ovrdval: Value=KOUTP_LRRawWhlSpeedTimeOut_flg_ovrdval
  VAPM_LRRawWhlSpeedVTimeOut_flg_Inproc : FVT_lib/outp/OverrideAndLimit  SystemSampleTime=-1  VariantActivationTime=update diagram  Latency=0  AutoFrameSizeCalculation=off
      link override Signal_Limit/_maxval: Value=KOUTP_LRRawWhlSpeedVTimeOut_flg_maxval
      link override Signal_Limit/_minval: Value=KOUTP_LRRawWhlSpeedVTimeOut_flg_minval
      link override Signal_Override/_ovrdflg: Value=KOUTP_LRRawWhlSpeedVTimeOut_flg_ovrdflg
      link override Signal_Override/_ovrdval: Value=KOUTP_LRRawWhlSpeedVTimeOut_flg_ovrdval
  VAPM_LRRawWhlSpeedV_flg_Inproc : FVT_lib/outp/OverrideAndLimit  SystemSampleTime=-1  VariantActivationTime=update diagram  Latency=0  AutoFrameSizeCalculation=off
      link override Signal_Limit/_maxval: Value=KOUTP_LRRawWhlSpeedV_flg_maxval
      link override Signal_Limit/_minval: Value=KOUTP_LRRawWhlSpeedV_flg_minval
      link override Signal_Override/_ovrdflg: Value=KOUTP_LRRawWhlSpeedV_flg_ovrdflg
      link override Signal_Override/_ovrdval: Value=KOUTP_LRRawWhlSpeedV_flg_ovrdval
  VAPM_LRRawWhlSpeed_kph_Inproc : FVT_lib/outp/OverrideAndLimit  SystemSampleTime=-1  VariantActivationTime=update diagram  Latency=0  AutoFrameSizeCalculation=off
      link override Signal_Limit/_maxval: Value=KOUTP_LRRawWhlSpeed_kph_maxval
      link override Signal_Limit/_minval: Value=KOUTP_LRRawWhlSpeed_kph_minval
      link override Signal_Override/_ovrdflg: Value=KOUTP_LRRawWhlSpeed_kph_ovrdflg
      link override Signal_Override/_ovrdval: Value=KOUTP_LRRawWhlSpeed_kph_ovrdval
  VAPM_LRWhlRotDirTimeOut_flg_Inproc : FVT_lib/outp/OverrideAndLimit  SystemSampleTime=-1  VariantActivationTime=update diagram  Latency=0  AutoFrameSizeCalculation=off
      link override Signal_Limit/_maxval: Value=KOUTP_LRWhlRotDirTimeOut_flg_maxval
      link override Signal_Limit/_minval: Value=KOUTP_LRWhlRotDirTimeOut_flg_minval
      link override Signal_Override/_ovrdflg: Value=KOUTP_LRWhlRotDirTimeOut_flg_ovrdflg
      link override Signal_Override/_ovrdval: Value=KOUTP_LRWhlRotDirTimeOut_flg_ovrdval
  VAPM_LRWhlRotDir_enum_Inproc : FVT_lib/outp/OverrideAndLimit  SystemSampleTime=-1  VariantActivationTime=update diagram  Latency=0  AutoFrameSizeCalculation=off
      link override Signal_Limit/_maxval: Value=KOUTP_LRWhlRotDir_enum_maxval
      link override Signal_Limit/_minval: Value=KOUTP_LRWhlRotDir_enum_minval
      link override Signal_Override/_ovrdflg: Value=KOUTP_LRWhlRotDir_enum_ovrdflg
      link override Signal_Override/_ovrdval: Value=KOUTP_LRWhlRotDir_enum_ovrdval
  VAPM_LatAccelTimeOut_flg_Inproc : FVT_lib/outp/OverrideAndLimit  SystemSampleTime=-1  VariantActivationTime=update diagram  Latency=0  AutoFrameSizeCalculation=off
      link override Signal_Limit/_maxval: Value=KOUTP_LatAccelTimeOut_flg_maxval
      link override Signal_Limit/_minval: Value=KOUTP_LatAccelTimeOut_flg_minval
      link override Signal_Override/_ovrdflg: Value=KOUTP_LatAccelTimeOut_flg_ovrdflg
      link override Signal_Override/_ovrdval: Value=KOUTP_LatAccelTimeOut_flg_ovrdval
  VAPM_LatAccelVTimeOut_flg_Inproc : FVT_lib/outp/OverrideAndLimit  SystemSampleTime=-1  VariantActivationTime=update diagram  Latency=0  AutoFrameSizeCalculation=off
      link override Signal_Limit/_maxval: Value=KOUTP_LatAccelVTimeOut_flg_maxval
      link override Signal_Limit/_minval: Value=KOUTP_LatAccelVTimeOut_flg_minval
      link override Signal_Override/_ovrdflg: Value=KOUTP_LatAccelVTimeOut_flg_ovrdflg
      link override Signal_Override/_ovrdval: Value=KOUTP_LatAccelVTimeOut_flg_ovrdval
  VAPM_LatAccelV_flg_Inproc : FVT_lib/outp/OverrideAndLimit  SystemSampleTime=-1  VariantActivationTime=update diagram  Latency=0  AutoFrameSizeCalculation=off
      link override Signal_Limit/_maxval: Value=KOUTP_LatAccelV_flg_maxval
      link override Signal_Limit/_minval: Value=KOUTP_LatAccelV_flg_minval
      link override Signal_Override/_ovrdflg: Value=KOUTP_LatAccelV_flg_ovrdflg
      link override Signal_Override/_ovrdval: Value=KOUTP_LatAccelV_flg_ovrdval
  VAPM_LatAccel_Gps_Inproc : FVT_lib/outp/OverrideAndLimit  SystemSampleTime=-1  VariantActivationTime=update diagram  Latency=0  AutoFrameSizeCalculation=off
      link override Signal_Limit/_maxval: Value=KOUTP_LatAccel_Gps_maxval
      link override Signal_Limit/_minval: Value=KOUTP_LatAccel_Gps_minval
      link override Signal_Override/_ovrdflg: Value=KOUTP_LatAccel_Gps_ovrdflg
      link override Signal_Override/_ovrdval: Value=KOUTP_LatAccel_Gps_ovrdval
  VAPM_LongAccelTimeOut_flg_Inproc : FVT_lib/outp/OverrideAndLimit  SystemSampleTime=-1  VariantActivationTime=update diagram  Latency=0  AutoFrameSizeCalculation=off
      link override Signal_Limit/_maxval: Value=KOUTP_LongAccelTimeOut_flg_maxval
      link override Signal_Limit/_minval: Value=KOUTP_LongAccelTimeOut_flg_minval
      link override Signal_Override/_ovrdflg: Value=KOUTP_LongAccelTimeOut_flg_ovrdflg
      link override Signal_Override/_ovrdval: Value=KOUTP_LongAccelTimeOut_flg_ovrdval
  VAPM_LongAccelVTimeOut_flg_Inproc : FVT_lib/outp/OverrideAndLimit  SystemSampleTime=-1  VariantActivationTime=update diagram  Latency=0  AutoFrameSizeCalculation=off
      link override Signal_Limit/_maxval: Value=KOUTP_LongAccelVTimeOut_flg_maxval
      link override Signal_Limit/_minval: Value=KOUTP_LongAccelVTimeOut_flg_minval
      link override Signal_Override/_ovrdflg: Value=KOUTP_LongAccelVTimeOut_flg_ovrdflg
      link override Signal_Override/_ovrdval: Value=KOUTP_LongAccelVTimeOut_flg_ovrdval
  VAPM_LongAccelV_flg_Inproc : FVT_lib/outp/OverrideAndLimit  SystemSampleTime=-1  VariantActivationTime=update diagram  Latency=0  AutoFrameSizeCalculation=off
      link override Signal_Limit/_maxval: Value=KOUTP_LongAccelV_flg_maxval
      link override Signal_Limit/_minval: Value=KOUTP_LongAccelV_flg_minval
      link override Signal_Override/_ovrdflg: Value=KOUTP_LongAccelV_flg_ovrdflg
      link override Signal_Override/_ovrdval: Value=KOUTP_LongAccelV_flg_ovrdval
  VAPM_LongAccel_Gps_Inproc : FVT_lib/outp/OverrideAndLimit  SystemSampleTime=-1  VariantActivationTime=update diagram  Latency=0  AutoFrameSizeCalculation=off
      link override Signal_Limit/_maxval: Value=KOUTP_LongAccel_Gps_maxval
      link override Signal_Limit/_minval: Value=KOUTP_LongAccel_Gps_minval
      link override Signal_Override/_ovrdflg: Value=KOUTP_LongAccel_Gps_ovrdflg
      link override Signal_Override/_ovrdval: Value=KOUTP_LongAccel_Gps_ovrdval
  VAPM_MCPressureTimeOut_flg_Inproc : FVT_lib/outp/OverrideAndLimit  SystemSampleTime=-1  VariantActivationTime=update diagram  Latency=0  AutoFrameSizeCalculation=off
      link override Signal_Limit/_maxval: Value=KOUTP_MCPressureTimeOut_flg_maxval
      link override Signal_Limit/_minval: Value=KOUTP_MCPressureTimeOut_flg_minval
      link override Signal_Override/_ovrdflg: Value=KOUTP_MCPressureTimeOut_flg_ovrdflg
      link override Signal_Override/_ovrdval: Value=KOUTP_MCPressureTimeOut_flg_ovrdval
  VAPM_MCPressureVTimeOut_flg_Inproc : FVT_lib/outp/OverrideAndLimit  SystemSampleTime=-1  VariantActivationTime=update diagram  Latency=0  AutoFrameSizeCalculation=off
      link override Signal_Limit/_maxval: Value=KOUTP_MCPressureVTimeOut_flg_maxval
      link override Signal_Limit/_minval: Value=KOUTP_MCPressureVTimeOut_flg_minval
      link override Signal_Override/_ovrdflg: Value=KOUTP_MCPressureVTimeOut_flg_ovrdflg
      link override Signal_Override/_ovrdval: Value=KOUTP_MCPressureVTimeOut_flg_ovrdval
  VAPM_MCPressureV_bar_Inproc : FVT_lib/outp/OverrideAndLimit  SystemSampleTime=-1  VariantActivationTime=update diagram  Latency=0  AutoFrameSizeCalculation=off
      link override Signal_Limit/_maxval: Value=KOUTP_MCPressureV_bar_maxval
      link override Signal_Limit/_minval: Value=KOUTP_MCPressureV_bar_minval
      link override Signal_Override/_ovrdflg: Value=KOUTP_MCPressureV_bar_ovrdflg
      link override Signal_Override/_ovrdval: Value=KOUTP_MCPressureV_bar_ovrdval
  VAPM_MCPressure_bar_Inproc : FVT_lib/outp/OverrideAndLimit  SystemSampleTime=-1  VariantActivationTime=update diagram  Latency=0  AutoFrameSizeCalculation=off
      link override Signal_Limit/_maxval: Value=KOUTP_MCPressure_bar_maxval
      link override Signal_Limit/_minval: Value=KOUTP_MCPressure_bar_minval
      link override Signal_Override/_ovrdflg: Value=KOUTP_MCPressure_bar_ovrdflg
      link override Signal_Override/_ovrdval: Value=KOUTP_MCPressure_bar_ovrdval
  VAPM_ModOperation_enum_Inproc : FVT_lib/outp/OverrideAndLimit  SystemSampleTime=-1  VariantActivationTime=update diagram  Latency=0  AutoFrameSizeCalculation=off
      link override Signal_Limit/_maxval: Value=KOUTP_ModOperation_enum_maxval
      link override Signal_Limit/_minval: Value=KOUTP_ModOperation_enum_minval
      link override Signal_Override/_ovrdflg: Value=KOUTP_ModOperation_enum_ovrdflg
      link override Signal_Override/_ovrdval: Value=KOUTP_ModOperation_enum_ovrdval
  VAPM_PASAFCL_enum_Inproc : FVT_lib/outp/OverrideAndLimit  SystemSampleTime=-1  VariantActivationTime=update diagram  Latency=0  AutoFrameSizeCalculation=off
      link override Signal_Limit/_maxval: Value=KOUTP_PASAFCL_enum_maxval
      link override Signal_Limit/_minval: Value=KOUTP_PASAFCL_enum_minval
      link override Signal_Override/_ovrdflg: Value=KOUTP_PASAFCL_enum_ovrdflg
      link override Signal_Override/_ovrdval: Value=KOUTP_PASAFCL_enum_ovrdval
  VAPM_PASAFCR_enum_Inproc : FVT_lib/outp/OverrideAndLimit  SystemSampleTime=-1  VariantActivationTime=update diagram  Latency=0  AutoFrameSizeCalculation=off
      link override Signal_Limit/_maxval: Value=KOUTP_PASAFCR_enum_maxval
      link override Signal_Limit/_minval: Value=KOUTP_PASAFCR_enum_minval
      link override Signal_Override/_ovrdflg: Value=KOUTP_PASAFCR_enum_ovrdflg
      link override Signal_Override/_ovrdval: Value=KOUTP_PASAFCR_enum_ovrdval
  VAPM_PASAFML_enum_Inproc : FVT_lib/outp/OverrideAndLimit  SystemSampleTime=-1  VariantActivationTime=update diagram  Latency=0  AutoFrameSizeCalculation=off
      link override Signal_Limit/_maxval: Value=KOUTP_PASAFML_enum_maxval
      link override Signal_Limit/_minval: Value=KOUTP_PASAFML_enum_minval
      link override Signal_Override/_ovrdflg: Value=KOUTP_PASAFML_enum_ovrdflg
      link override Signal_Override/_ovrdval: Value=KOUTP_PASAFML_enum_ovrdval
  VAPM_PASAFMR_enum_Inproc : FVT_lib/outp/OverrideAndLimit  SystemSampleTime=-1  VariantActivationTime=update diagram  Latency=0  AutoFrameSizeCalculation=off
      link override Signal_Limit/_maxval: Value=KOUTP_PASAFMR_enum_maxval
      link override Signal_Limit/_minval: Value=KOUTP_PASAFMR_enum_minval
      link override Signal_Override/_ovrdflg: Value=KOUTP_PASAFMR_enum_ovrdflg
      link override Signal_Override/_ovrdval: Value=KOUTP_PASAFMR_enum_ovrdval
  VAPM_PASARCL_enum_Inproc : FVT_lib/outp/OverrideAndLimit  SystemSampleTime=-1  VariantActivationTime=update diagram  Latency=0  AutoFrameSizeCalculation=off
      link override Signal_Limit/_maxval: Value=KOUTP_PASARCL_enum_maxval
      link override Signal_Limit/_minval: Value=KOUTP_PASARCL_enum_minval
      link override Signal_Override/_ovrdflg: Value=KOUTP_PASARCL_enum_ovrdflg
      link override Signal_Override/_ovrdval: Value=KOUTP_PASARCL_enum_ovrdval
  VAPM_PASARCR_enum_Inproc : FVT_lib/outp/OverrideAndLimit  SystemSampleTime=-1  VariantActivationTime=update diagram  Latency=0  AutoFrameSizeCalculation=off
      link override Signal_Limit/_maxval: Value=KOUTP_PASARCR_enum_maxval
      link override Signal_Limit/_minval: Value=KOUTP_PASARCR_enum_minval
      link override Signal_Override/_ovrdflg: Value=KOUTP_PASARCR_enum_ovrdflg
      link override Signal_Override/_ovrdval: Value=KOUTP_PASARCR_enum_ovrdval
  VAPM_PASARML_enum_Inproc : FVT_lib/outp/OverrideAndLimit  SystemSampleTime=-1  VariantActivationTime=update diagram  Latency=0  AutoFrameSizeCalculation=off
      link override Signal_Limit/_maxval: Value=KOUTP_PASARML_enum_maxval
      link override Signal_Limit/_minval: Value=KOUTP_PASARML_enum_minval
      link override Signal_Override/_ovrdflg: Value=KOUTP_PASARML_enum_ovrdflg
      link override Signal_Override/_ovrdval: Value=KOUTP_PASARML_enum_ovrdval
  VAPM_PASARMR_enum_Inproc : FVT_lib/outp/OverrideAndLimit  SystemSampleTime=-1  VariantActivationTime=update diagram  Latency=0  AutoFrameSizeCalculation=off
      link override Signal_Limit/_maxval: Value=KOUTP_PASARMR_enum_maxval
      link override Signal_Limit/_minval: Value=KOUTP_PASARMR_enum_minval
      link override Signal_Override/_ovrdflg: Value=KOUTP_PASARMR_enum_ovrdflg
      link override Signal_Override/_ovrdval: Value=KOUTP_PASARMR_enum_ovrdval
  VAPM_PASDFCL_cm_Inproc : FVT_lib/outp/OverrideAndLimit  SystemSampleTime=-1  VariantActivationTime=update diagram  Latency=0  AutoFrameSizeCalculation=off
      link override Signal_Limit/_maxval: Value=KOUTP_PASDFCL_cm_maxval
      link override Signal_Limit/_minval: Value=KOUTP_PASDFCL_cm_minval
      link override Signal_Override/_ovrdflg: Value=KOUTP_PASDFCL_cm_ovrdflg
      link override Signal_Override/_ovrdval: Value=KOUTP_PASDFCL_cm_ovrdval
  VAPM_PASDFCR_cm_Inproc : FVT_lib/outp/OverrideAndLimit  SystemSampleTime=-1  VariantActivationTime=update diagram  Latency=0  AutoFrameSizeCalculation=off
      link override Signal_Limit/_maxval: Value=KOUTP_PASDFCR_cm_maxval
      link override Signal_Limit/_minval: Value=KOUTP_PASDFCR_cm_minval
      link override Signal_Override/_ovrdflg: Value=KOUTP_PASDFCR_cm_ovrdflg
      link override Signal_Override/_ovrdval: Value=KOUTP_PASDFCR_cm_ovrdval
  VAPM_PASDFML_cm_Inproc : FVT_lib/outp/OverrideAndLimit  SystemSampleTime=-1  VariantActivationTime=update diagram  Latency=0  AutoFrameSizeCalculation=off
      link override Signal_Limit/_maxval: Value=KOUTP_PASDFML_cm_maxval
      link override Signal_Limit/_minval: Value=KOUTP_PASDFML_cm_minval
      link override Signal_Override/_ovrdflg: Value=KOUTP_PASDFML_cm_ovrdflg
      link override Signal_Override/_ovrdval: Value=KOUTP_PASDFML_cm_ovrdval
  VAPM_PASDFMR_cm_Inproc : FVT_lib/outp/OverrideAndLimit  SystemSampleTime=-1  VariantActivationTime=update diagram  Latency=0  AutoFrameSizeCalculation=off
      link override Signal_Limit/_maxval: Value=KOUTP_PASDFMR_cm_maxval
      link override Signal_Limit/_minval: Value=KOUTP_PASDFMR_cm_minval
      link override Signal_Override/_ovrdflg: Value=KOUTP_PASDFMR_cm_ovrdflg
      link override Signal_Override/_ovrdval: Value=KOUTP_PASDFMR_cm_ovrdval
  VAPM_PASDRCL_cm_Inproc : FVT_lib/outp/OverrideAndLimit  SystemSampleTime=-1  VariantActivationTime=update diagram  Latency=0  AutoFrameSizeCalculation=off
      link override Signal_Limit/_maxval: Value=KOUTP_PASDRCL_cm_maxval
      link override Signal_Limit/_minval: Value=KOUTP_PASDRCL_cm_minval
      link override Signal_Override/_ovrdflg: Value=KOUTP_PASDRCL_cm_ovrdflg
      link override Signal_Override/_ovrdval: Value=KOUTP_PASDRCL_cm_ovrdval
  VAPM_PASDRCR_cm_Inproc : FVT_lib/outp/OverrideAndLimit  SystemSampleTime=-1  VariantActivationTime=update diagram  Latency=0  AutoFrameSizeCalculation=off
      link override Signal_Limit/_maxval: Value=KOUTP_PASDRCR_cm_maxval
      link override Signal_Limit/_minval: Value=KOUTP_PASDRCR_cm_minval
      link override Signal_Override/_ovrdflg: Value=KOUTP_PASDRCR_cm_ovrdflg
      link override Signal_Override/_ovrdval: Value=KOUTP_PASDRCR_cm_ovrdval
  VAPM_PASDRML_cm_Inproc : FVT_lib/outp/OverrideAndLimit  SystemSampleTime=-1  VariantActivationTime=update diagram  Latency=0  AutoFrameSizeCalculation=off
      link override Signal_Limit/_maxval: Value=KOUTP_PASDRML_cm_maxval
      link override Signal_Limit/_minval: Value=KOUTP_PASDRML_cm_minval
      link override Signal_Override/_ovrdflg: Value=KOUTP_PASDRML_cm_ovrdflg
      link override Signal_Override/_ovrdval: Value=KOUTP_PASDRML_cm_ovrdval
  VAPM_PASDRMR_cm_Inproc : FVT_lib/outp/OverrideAndLimit  SystemSampleTime=-1  VariantActivationTime=update diagram  Latency=0  AutoFrameSizeCalculation=off
      link override Signal_Limit/_maxval: Value=KOUTP_PASDRMR_cm_maxval
      link override Signal_Limit/_minval: Value=KOUTP_PASDRMR_cm_minval
      link override Signal_Override/_ovrdflg: Value=KOUTP_PASDRMR_cm_ovrdflg
      link override Signal_Override/_ovrdval: Value=KOUTP_PASDRMR_cm_ovrdval
  VAPM_RFPulseCountTimeOut_flg_Inproc : FVT_lib/outp/OverrideAndLimit  SystemSampleTime=-1  VariantActivationTime=update diagram  Latency=0  AutoFrameSizeCalculation=off
      link override Signal_Limit/_maxval: Value=KOUTP_RFPulseCountTimeOut_flg_maxval
      link override Signal_Limit/_minval: Value=KOUTP_RFPulseCountTimeOut_flg_minval
      link override Signal_Override/_ovrdflg: Value=KOUTP_RFPulseCountTimeOut_flg_ovrdflg
      link override Signal_Override/_ovrdval: Value=KOUTP_RFPulseCountTimeOut_flg_ovrdval
  VAPM_RFPulseCountVTimeOut_flg_Inproc : FVT_lib/outp/OverrideAndLimit  SystemSampleTime=-1  VariantActivationTime=update diagram  Latency=0  AutoFrameSizeCalculation=off
      link override Signal_Limit/_maxval: Value=KOUTP_RFPulseCountVTimeOut_flg_maxval
      link override Signal_Limit/_minval: Value=KOUTP_RFPulseCountVTimeOut_flg_minval
      link override Signal_Override/_ovrdflg: Value=KOUTP_RFPulseCountVTimeOut_flg_ovrdflg
      link override Signal_Override/_ovrdval: Value=KOUTP_RFPulseCountVTimeOut_flg_ovrdval
  VAPM_RFPulseCountV_flg_Inproc : FVT_lib/outp/OverrideAndLimit  SystemSampleTime=-1  VariantActivationTime=update diagram  Latency=0  AutoFrameSizeCalculation=off
      link override Signal_Limit/_maxval: Value=KOUTP_RFPulseCountV_flg_maxval
      link override Signal_Limit/_minval: Value=KOUTP_RFPulseCountV_flg_minval
      link override Signal_Override/_ovrdflg: Value=KOUTP_RFPulseCountV_flg_ovrdflg
      link override Signal_Override/_ovrdval: Value=KOUTP_RFPulseCountV_flg_ovrdval
  VAPM_RFPulseCount_enum_Inproc : FVT_lib/outp/OverrideAndLimit  SystemSampleTime=-1  VariantActivationTime=update diagram  Latency=0  AutoFrameSizeCalculation=off
      link override Signal_Limit/_maxval: Value=KOUTP_RFPulseCount_enum_maxval
      link override Signal_Limit/_minval: Value=KOUTP_RFPulseCount_enum_minval
      link override Signal_Override/_ovrdflg: Value=KOUTP_RFPulseCount_enum_ovrdflg
      link override Signal_Override/_ovrdval: Value=KOUTP_RFPulseCount_enum_ovrdval
  VAPM_RFRawWhlSpeedTimeOut_flg_Inproc : FVT_lib/outp/OverrideAndLimit  SystemSampleTime=-1  VariantActivationTime=update diagram  Latency=0  AutoFrameSizeCalculation=off
      link override Signal_Limit/_maxval: Value=KOUTP_RFRawWhlSpeedTimeOut_flg_maxval
      link override Signal_Limit/_minval: Value=KOUTP_RFRawWhlSpeedTimeOut_flg_minval
      link override Signal_Override/_ovrdflg: Value=KOUTP_RFRawWhlSpeedTimeOut_flg_ovrdflg
      link override Signal_Override/_ovrdval: Value=KOUTP_RFRawWhlSpeedTimeOut_flg_ovrdval
  VAPM_RFRawWhlSpeedVTimeOut_flg_Inproc : FVT_lib/outp/OverrideAndLimit  SystemSampleTime=-1  VariantActivationTime=update diagram  Latency=0  AutoFrameSizeCalculation=off
      link override Signal_Limit/_maxval: Value=KOUTP_RFRawWhlSpeedVTimeOut_flg_maxval
      link override Signal_Limit/_minval: Value=KOUTP_RFRawWhlSpeedVTimeOut_flg_minval
      link override Signal_Override/_ovrdflg: Value=KOUTP_RFRawWhlSpeedVTimeOut_flg_ovrdflg
      link override Signal_Override/_ovrdval: Value=KOUTP_RFRawWhlSpeedVTimeOut_flg_ovrdval
  VAPM_RFRawWhlSpeedV_flg_Inproc : FVT_lib/outp/OverrideAndLimit  SystemSampleTime=-1  VariantActivationTime=update diagram  Latency=0  AutoFrameSizeCalculation=off
      link override Signal_Limit/_maxval: Value=KOUTP_RFRawWhlSpeedV_flg_maxval
      link override Signal_Limit/_minval: Value=KOUTP_RFRawWhlSpeedV_flg_minval
      link override Signal_Override/_ovrdflg: Value=KOUTP_RFRawWhlSpeedV_flg_ovrdflg
      link override Signal_Override/_ovrdval: Value=KOUTP_RFRawWhlSpeedV_flg_ovrdval
  VAPM_RFRawWhlSpeed_kph_Inproc : FVT_lib/outp/OverrideAndLimit  SystemSampleTime=-1  VariantActivationTime=update diagram  Latency=0  AutoFrameSizeCalculation=off
      link override Signal_Limit/_maxval: Value=KOUTP_RFRawWhlSpeed_kph_maxval
      link override Signal_Limit/_minval: Value=KOUTP_RFRawWhlSpeed_kph_minval
      link override Signal_Override/_ovrdflg: Value=KOUTP_RFRawWhlSpeed_kph_ovrdflg
      link override Signal_Override/_ovrdval: Value=KOUTP_RFRawWhlSpeed_kph_ovrdval
  VAPM_RFWhlRotDirTimeOut_flg_Inproc : FVT_lib/outp/OverrideAndLimit  SystemSampleTime=-1  VariantActivationTime=update diagram  Latency=0  AutoFrameSizeCalculation=off
      link override Signal_Limit/_maxval: Value=KOUTP_RFWhlRotDirTimeOut_flg_maxval
      link override Signal_Limit/_minval: Value=KOUTP_RFWhlRotDirTimeOut_flg_minval
      link override Signal_Override/_ovrdflg: Value=KOUTP_RFWhlRotDirTimeOut_flg_ovrdflg
      link override Signal_Override/_ovrdval: Value=KOUTP_RFWhlRotDirTimeOut_flg_ovrdval
  VAPM_RFWhlRotDir_enum_Inproc : FVT_lib/outp/OverrideAndLimit  SystemSampleTime=-1  VariantActivationTime=update diagram  Latency=0  AutoFrameSizeCalculation=off
      link override Signal_Limit/_maxval: Value=KOUTP_RFWhlRotDir_enum_maxval
      link override Signal_Limit/_minval: Value=KOUTP_RFWhlRotDir_enum_minval
      link override Signal_Override/_ovrdflg: Value=KOUTP_RFWhlRotDir_enum_ovrdflg
      link override Signal_Override/_ovrdval: Value=KOUTP_RFWhlRotDir_enum_ovrdval
  VAPM_RRPulseCountTimeOut_flg_Inproc : FVT_lib/outp/OverrideAndLimit  SystemSampleTime=-1  VariantActivationTime=update diagram  Latency=0  AutoFrameSizeCalculation=off
      link override Signal_Limit/_maxval: Value=KOUTP_RRPulseCountTimeOut_flg_maxval
      link override Signal_Limit/_minval: Value=KOUTP_RRPulseCountTimeOut_flg_minval
      link override Signal_Override/_ovrdflg: Value=KOUTP_RRPulseCountTimeOut_flg_ovrdflg
      link override Signal_Override/_ovrdval: Value=KOUTP_RRPulseCountTimeOut_flg_ovrdval
  VAPM_RRPulseCountVTimeOut_flg_Inproc : FVT_lib/outp/OverrideAndLimit  SystemSampleTime=-1  VariantActivationTime=update diagram  Latency=0  AutoFrameSizeCalculation=off
      link override Signal_Limit/_maxval: Value=KOUTP_RRPulseCountVTimeOut_flg_maxval
      link override Signal_Limit/_minval: Value=KOUTP_RRPulseCountVTimeOut_flg_minval
      link override Signal_Override/_ovrdflg: Value=KOUTP_RRPulseCountVTimeOut_flg_ovrdflg
      link override Signal_Override/_ovrdval: Value=KOUTP_RRPulseCountVTimeOut_flg_ovrdval
  VAPM_RRPulseCountV_flg_Inproc : FVT_lib/outp/OverrideAndLimit  SystemSampleTime=-1  VariantActivationTime=update diagram  Latency=0  AutoFrameSizeCalculation=off
      link override Signal_Limit/_maxval: Value=KOUTP_RRPulseCountV_flg_maxval
      link override Signal_Limit/_minval: Value=KOUTP_RRPulseCountV_flg_minval
      link override Signal_Override/_ovrdflg: Value=KOUTP_RRPulseCountV_flg_ovrdflg
      link override Signal_Override/_ovrdval: Value=KOUTP_RRPulseCountV_flg_ovrdval
  VAPM_RRPulseCount_enum_Inproc : FVT_lib/outp/OverrideAndLimit  SystemSampleTime=-1  VariantActivationTime=update diagram  Latency=0  AutoFrameSizeCalculation=off
      link override Signal_Limit/_maxval: Value=KOUTP_RRPulseCount_enum_maxval
      link override Signal_Limit/_minval: Value=KOUTP_RRPulseCount_enum_minval
      link override Signal_Override/_ovrdflg: Value=KOUTP_RRPulseCount_enum_ovrdflg
      link override Signal_Override/_ovrdval: Value=KOUTP_RRPulseCount_enum_ovrdval
  VAPM_RRRawWhlSpeedTimeOut_flg_Inproc : FVT_lib/outp/OverrideAndLimit  SystemSampleTime=-1  VariantActivationTime=update diagram  Latency=0  AutoFrameSizeCalculation=off
      link override Signal_Limit/_maxval: Value=KOUTP_RRRawWhlSpeedTimeOut_flg_maxval
      link override Signal_Limit/_minval: Value=KOUTP_RRRawWhlSpeedTimeOut_flg_minval
      link override Signal_Override/_ovrdflg: Value=KOUTP_RRRawWhlSpeedTimeOut_flg_ovrdflg
      link override Signal_Override/_ovrdval: Value=KOUTP_RRRawWhlSpeedTimeOut_flg_ovrdval
  VAPM_RRRawWhlSpeedVTimeOut_flg_Inproc : FVT_lib/outp/OverrideAndLimit  SystemSampleTime=-1  VariantActivationTime=update diagram  Latency=0  AutoFrameSizeCalculation=off
      link override Signal_Limit/_maxval: Value=KOUTP_RRRawWhlSpeedVTimeOut_flg_maxval
      link override Signal_Limit/_minval: Value=KOUTP_RRRawWhlSpeedVTimeOut_flg_minval
      link override Signal_Override/_ovrdflg: Value=KOUTP_RRRawWhlSpeedVTimeOut_flg_ovrdflg
      link override Signal_Override/_ovrdval: Value=KOUTP_RRRawWhlSpeedVTimeOut_flg_ovrdval
  VAPM_RRRawWhlSpeedV_flg_Inproc : FVT_lib/outp/OverrideAndLimit  SystemSampleTime=-1  VariantActivationTime=update diagram  Latency=0  AutoFrameSizeCalculation=off
      link override Signal_Limit/_maxval: Value=KOUTP_RRRawWhlSpeedV_flg_maxval
      link override Signal_Limit/_minval: Value=KOUTP_RRRawWhlSpeedV_flg_minval
      link override Signal_Override/_ovrdflg: Value=KOUTP_RRRawWhlSpeedV_flg_ovrdflg
      link override Signal_Override/_ovrdval: Value=KOUTP_RRRawWhlSpeedV_flg_ovrdval
  VAPM_RRRawWhlSpeed_kph_Inproc : FVT_lib/outp/OverrideAndLimit  SystemSampleTime=-1  VariantActivationTime=update diagram  Latency=0  AutoFrameSizeCalculation=off
      link override Signal_Limit/_maxval: Value=KOUTP_RRRawWhlSpeed_kph_maxval
      link override Signal_Limit/_minval: Value=KOUTP_RRRawWhlSpeed_kph_minval
      link override Signal_Override/_ovrdflg: Value=KOUTP_RRRawWhlSpeed_kph_ovrdflg
      link override Signal_Override/_ovrdval: Value=KOUTP_RRRawWhlSpeed_kph_ovrdval
  VAPM_RRWhlRotDirTimeOut_flg_Inproc : FVT_lib/outp/OverrideAndLimit  SystemSampleTime=-1  VariantActivationTime=update diagram  Latency=0  AutoFrameSizeCalculation=off
      link override Signal_Limit/_maxval: Value=KOUTP_RRWhlRotDirTimeOut_flg_maxval
      link override Signal_Limit/_minval: Value=KOUTP_RRWhlRotDirTimeOut_flg_minval
      link override Signal_Override/_ovrdflg: Value=KOUTP_RRWhlRotDirTimeOut_flg_ovrdflg
      link override Signal_Override/_ovrdval: Value=KOUTP_RRWhlRotDirTimeOut_flg_ovrdval
  VAPM_RRWhlRotDir_enum_Inproc : FVT_lib/outp/OverrideAndLimit  SystemSampleTime=-1  VariantActivationTime=update diagram  Latency=0  AutoFrameSizeCalculation=off
      link override Signal_Limit/_maxval: Value=KOUTP_RRWhlRotDir_enum_maxval
      link override Signal_Limit/_minval: Value=KOUTP_RRWhlRotDir_enum_minval
      link override Signal_Override/_ovrdflg: Value=KOUTP_RRWhlRotDir_enum_ovrdflg
      link override Signal_Override/_ovrdval: Value=KOUTP_RRWhlRotDir_enum_ovrdval
  VAPM_SASAngleTimeOut_flg_Inproc : FVT_lib/outp/OverrideAndLimit  SystemSampleTime=-1  VariantActivationTime=update diagram  Latency=0  AutoFrameSizeCalculation=off
      link override Signal_Limit/_maxval: Value=KOUTP_SASAngleTimeOut_flg_maxval
      link override Signal_Limit/_minval: Value=KOUTP_SASAngleTimeOut_flg_minval
      link override Signal_Override/_ovrdflg: Value=KOUTP_SASAngleTimeOut_flg_ovrdflg
      link override Signal_Override/_ovrdval: Value=KOUTP_SASAngleTimeOut_flg_ovrdval
  VAPM_SASAngle_Deg_Inproc : FVT_lib/outp/OverrideAndLimit  SystemSampleTime=-1  VariantActivationTime=update diagram  Latency=0  AutoFrameSizeCalculation=off
      link override Signal_Limit/_maxval: Value=KOUTP_SASAngle_Deg_maxval
      link override Signal_Limit/_minval: Value=KOUTP_SASAngle_Deg_minval
      link override Signal_Override/_ovrdflg: Value=KOUTP_SASAngle_Deg_ovrdflg
      link override Signal_Override/_ovrdval: Value=KOUTP_SASAngle_Deg_ovrdval
  VAPM_SASCALTimeOut_flg_Inproc : FVT_lib/outp/OverrideAndLimit  SystemSampleTime=-1  VariantActivationTime=update diagram  Latency=0  AutoFrameSizeCalculation=off
      link override Signal_Limit/_maxval: Value=KOUTP_SASCALTimeOut_flg_maxval
      link override Signal_Limit/_minval: Value=KOUTP_SASCALTimeOut_flg_minval
      link override Signal_Override/_ovrdflg: Value=KOUTP_SASCALTimeOut_flg_ovrdflg
      link override Signal_Override/_ovrdval: Value=KOUTP_SASCALTimeOut_flg_ovrdval
  VAPM_SASCAL_flg_Inproc : FVT_lib/outp/OverrideAndLimit  SystemSampleTime=-1  VariantActivationTime=update diagram  Latency=0  AutoFrameSizeCalculation=off
      link override Signal_Limit/_maxval: Value=KOUTP_SASCAL_flg_maxval
      link override Signal_Limit/_minval: Value=KOUTP_SASCAL_flg_minval
      link override Signal_Override/_ovrdflg: Value=KOUTP_SASCAL_flg_ovrdflg
      link override Signal_Override/_ovrdval: Value=KOUTP_SASCAL_flg_ovrdval
  VAPM_SASSpeedTimeOut_flg_Inproc : FVT_lib/outp/OverrideAndLimit  SystemSampleTime=-1  VariantActivationTime=update diagram  Latency=0  AutoFrameSizeCalculation=off
      link override Signal_Limit/_maxval: Value=KOUTP_SASSpeedTimeOut_flg_maxval
      link override Signal_Limit/_minval: Value=KOUTP_SASSpeedTimeOut_flg_minval
      link override Signal_Override/_ovrdflg: Value=KOUTP_SASSpeedTimeOut_flg_ovrdflg
      link override Signal_Override/_ovrdval: Value=KOUTP_SASSpeedTimeOut_flg_ovrdval
  VAPM_SASSpeedValidTimeOut_flg_Inproc : FVT_lib/outp/OverrideAndLimit  SystemSampleTime=-1  VariantActivationTime=update diagram  Latency=0  AutoFrameSizeCalculation=off
      link override Signal_Limit/_maxval: Value=KOUTP_SASSpeedValidTimeOut_flg_maxval
      link override Signal_Limit/_minval: Value=KOUTP_SASSpeedValidTimeOut_flg_minval
      link override Signal_Override/_ovrdflg: Value=KOUTP_SASSpeedValidTimeOut_flg_ovrdflg
      link override Signal_Override/_ovrdval: Value=KOUTP_SASSpeedValidTimeOut_flg_ovrdval
  VAPM_SASSpeedValid_flg_Inproc : FVT_lib/outp/OverrideAndLimit  SystemSampleTime=-1  VariantActivationTime=update diagram  Latency=0  AutoFrameSizeCalculation=off
      link override Signal_Limit/_maxval: Value=KOUTP_SASSpeedValid_flg_maxval
      link override Signal_Limit/_minval: Value=KOUTP_SASSpeedValid_flg_minval
      link override Signal_Override/_ovrdflg: Value=KOUTP_SASSpeedValid_flg_ovrdflg
      link override Signal_Override/_ovrdval: Value=KOUTP_SASSpeedValid_flg_ovrdval
  VAPM_SASSpeed_degps_Inproc : FVT_lib/outp/OverrideAndLimit  SystemSampleTime=-1  VariantActivationTime=update diagram  Latency=0  AutoFrameSizeCalculation=off
      link override Signal_Limit/_maxval: Value=KOUTP_SASSpeed_degps_maxval
      link override Signal_Limit/_minval: Value=KOUTP_SASSpeed_degps_minval
      link override Signal_Override/_ovrdflg: Value=KOUTP_SASSpeed_degps_ovrdflg
      link override Signal_Override/_ovrdval: Value=KOUTP_SASSpeed_degps_ovrdval
  VAPM_SASVTimeOut_flg_Inproc : FVT_lib/outp/OverrideAndLimit  SystemSampleTime=-1  VariantActivationTime=update diagram  Latency=0  AutoFrameSizeCalculation=off
      link override Signal_Limit/_maxval: Value=KOUTP_SASVTimeOut_flg_maxval
      link override Signal_Limit/_minval: Value=KOUTP_SASVTimeOut_flg_minval
      link override Signal_Override/_ovrdflg: Value=KOUTP_SASVTimeOut_flg_ovrdflg
      link override Signal_Override/_ovrdval: Value=KOUTP_SASVTimeOut_flg_ovrdval
  VAPM_SASV_flg_Inproc : FVT_lib/outp/OverrideAndLimit  SystemSampleTime=-1  VariantActivationTime=update diagram  Latency=0  AutoFrameSizeCalculation=off
      link override Signal_Limit/_maxval: Value=KOUTP_SASV_flg_maxval
      link override Signal_Limit/_minval: Value=KOUTP_SASV_flg_minval
      link override Signal_Override/_ovrdflg: Value=KOUTP_SASV_flg_ovrdflg
      link override Signal_Override/_ovrdval: Value=KOUTP_SASV_flg_ovrdval
  VAPM_SNSRLayout_enum_Inproc : FVT_lib/outp/OverrideAndLimit  SystemSampleTime=-1  VariantActivationTime=update diagram  Latency=0  AutoFrameSizeCalculation=off
      link override Signal_Limit/_maxval: Value=KOUTP_SNSRLayout_enum_maxval
      link override Signal_Limit/_minval: Value=KOUTP_SNSRLayout_enum_minval
      link override Signal_Override/_ovrdflg: Value=KOUTP_SNSRLayout_enum_ovrdflg
      link override Signal_Override/_ovrdval: Value=KOUTP_SNSRLayout_enum_ovrdval
  VAPM_ShifterHandleCmdTimeOut_flg_Inproc : FVT_lib/outp/OverrideAndLimit  SystemSampleTime=-1  VariantActivationTime=update diagram  Latency=0  AutoFrameSizeCalculation=off
      link override Signal_Limit/_maxval: Value=KOUTP_ShifterHandleCmdTimeOut_flg_maxval
      link override Signal_Limit/_minval: Value=KOUTP_ShifterHandleCmdTimeOut_flg_minval
      link override Signal_Override/_ovrdflg: Value=KOUTP_ShifterHandleCmdTimeOut_flg_ovrdflg
      link override Signal_Override/_ovrdval: Value=KOUTP_ShifterHandleCmdTimeOut_flg_ovrdval
  VAPM_ShifterHandleCmd_enum_Inproc : FVT_lib/outp/OverrideAndLimit  SystemSampleTime=-1  VariantActivationTime=update diagram  Latency=0  AutoFrameSizeCalculation=off
      link override Signal_Limit/_maxval: Value=KOUTP_ShifterHandleCmd_enum_maxval
      link override Signal_Limit/_minval: Value=KOUTP_ShifterHandleCmd_enum_minval
      link override Signal_Override/_ovrdflg: Value=KOUTP_ShifterHandleCmd_enum_ovrdflg
      link override Signal_Override/_ovrdval: Value=KOUTP_ShifterHandleCmd_enum_ovrdval
  VAPM_StaFSya_flg_Inproc : FVT_lib/outp/OverrideAndLimit  SystemSampleTime=-1  VariantActivationTime=update diagram  Latency=0  AutoFrameSizeCalculation=off
      link override Signal_Limit/_maxval: Value=KOUTP_StaFSya_flg_maxval
      link override Signal_Limit/_minval: Value=KOUTP_StaFSya_flg_minval
      link override Signal_Override/_ovrdflg: Value=KOUTP_StaFSya_flg_ovrdflg
      link override Signal_Override/_ovrdval: Value=KOUTP_StaFSya_flg_ovrdval
  VAPM_TCSActiveTimeOut_flg_Inproc : FVT_lib/outp/OverrideAndLimit  SystemSampleTime=-1  VariantActivationTime=update diagram  Latency=0  AutoFrameSizeCalculation=off
      link override Signal_Limit/_maxval: Value=KOUTP_TCSActiveTimeOut_flg_maxval
      link override Signal_Limit/_minval: Value=KOUTP_TCSActiveTimeOut_flg_minval
      link override Signal_Override/_ovrdflg: Value=KOUTP_TCSActiveTimeOut_flg_ovrdflg
      link override Signal_Override/_ovrdval: Value=KOUTP_TCSActiveTimeOut_flg_ovrdval
  VAPM_TCSActive_flg_Inproc : FVT_lib/outp/OverrideAndLimit  SystemSampleTime=-1  VariantActivationTime=update diagram  Latency=0  AutoFrameSizeCalculation=off
      link override Signal_Limit/_maxval: Value=KOUTP_TCSActive_flg_maxval
      link override Signal_Limit/_minval: Value=KOUTP_TCSActive_flg_minval
      link override Signal_Override/_ovrdflg: Value=KOUTP_TCSActive_flg_ovrdflg
      link override Signal_Override/_ovrdval: Value=KOUTP_TCSActive_flg_ovrdval
  VAPM_USSStaFCL_flg_Inproc : FVT_lib/outp/OverrideAndLimit  SystemSampleTime=-1  VariantActivationTime=update diagram  Latency=0  AutoFrameSizeCalculation=off
      link override Signal_Limit/_maxval: Value=KOUTP_USSStaFCL_flg_maxval
      link override Signal_Limit/_minval: Value=KOUTP_USSStaFCL_flg_minval
      link override Signal_Override/_ovrdflg: Value=KOUTP_USSStaFCL_flg_ovrdflg
      link override Signal_Override/_ovrdval: Value=KOUTP_USSStaFCL_flg_ovrdval
  VAPM_USSStaFCR_flg_Inproc : FVT_lib/outp/OverrideAndLimit  SystemSampleTime=-1  VariantActivationTime=update diagram  Latency=0  AutoFrameSizeCalculation=off
      link override Signal_Limit/_maxval: Value=KOUTP_USSStaFCR_flg_maxval
      link override Signal_Limit/_minval: Value=KOUTP_USSStaFCR_flg_minval
      link override Signal_Override/_ovrdflg: Value=KOUTP_USSStaFCR_flg_ovrdflg
      link override Signal_Override/_ovrdval: Value=KOUTP_USSStaFCR_flg_ovrdval
  VAPM_USSStaFLL_flg_Inproc : FVT_lib/outp/OverrideAndLimit  SystemSampleTime=-1  VariantActivationTime=update diagram  Latency=0  AutoFrameSizeCalculation=off
      link override Signal_Limit/_maxval: Value=KOUTP_USSStaFLL_flg_maxval
      link override Signal_Limit/_minval: Value=KOUTP_USSStaFLL_flg_minval
      link override Signal_Override/_ovrdflg: Value=KOUTP_USSStaFLL_flg_ovrdflg
      link override Signal_Override/_ovrdval: Value=KOUTP_USSStaFLL_flg_ovrdval
  VAPM_USSStaFLR_flg_Inproc : FVT_lib/outp/OverrideAndLimit  SystemSampleTime=-1  VariantActivationTime=update diagram  Latency=0  AutoFrameSizeCalculation=off
      link override Signal_Limit/_maxval: Value=KOUTP_USSStaFLR_flg_maxval
      link override Signal_Limit/_minval: Value=KOUTP_USSStaFLR_flg_minval
      link override Signal_Override/_ovrdflg: Value=KOUTP_USSStaFLR_flg_ovrdflg
      link override Signal_Override/_ovrdval: Value=KOUTP_USSStaFLR_flg_ovrdval
  VAPM_USSStaFML_flg_Inproc : FVT_lib/outp/OverrideAndLimit  SystemSampleTime=-1  VariantActivationTime=update diagram  Latency=0  AutoFrameSizeCalculation=off
      link override Signal_Limit/_maxval: Value=KOUTP_USSStaFML_flg_maxval
      link override Signal_Limit/_minval: Value=KOUTP_USSStaFML_flg_minval
      link override Signal_Override/_ovrdflg: Value=KOUTP_USSStaFML_flg_ovrdflg
      link override Signal_Override/_ovrdval: Value=KOUTP_USSStaFML_flg_ovrdval
  VAPM_USSStaFMR_flg_Inproc : FVT_lib/outp/OverrideAndLimit  SystemSampleTime=-1  VariantActivationTime=update diagram  Latency=0  AutoFrameSizeCalculation=off
      link override Signal_Limit/_maxval: Value=KOUTP_USSStaFMR_flg_maxval
      link override Signal_Limit/_minval: Value=KOUTP_USSStaFMR_flg_minval
      link override Signal_Override/_ovrdflg: Value=KOUTP_USSStaFMR_flg_ovrdflg
      link override Signal_Override/_ovrdval: Value=KOUTP_USSStaFMR_flg_ovrdval
  VAPM_USSStaRCL_flg_Inproc : FVT_lib/outp/OverrideAndLimit  SystemSampleTime=-1  VariantActivationTime=update diagram  Latency=0  AutoFrameSizeCalculation=off
      link override Signal_Limit/_maxval: Value=KOUTP_USSStaRCL_flg_maxval
      link override Signal_Limit/_minval: Value=KOUTP_USSStaRCL_flg_minval
      link override Signal_Override/_ovrdflg: Value=KOUTP_USSStaRCL_flg_ovrdflg
      link override Signal_Override/_ovrdval: Value=KOUTP_USSStaRCL_flg_ovrdval
  VAPM_USSStaRCR_flg_Inproc : FVT_lib/outp/OverrideAndLimit  SystemSampleTime=-1  VariantActivationTime=update diagram  Latency=0  AutoFrameSizeCalculation=off
      link override Signal_Limit/_maxval: Value=KOUTP_USSStaRCR_flg_maxval
      link override Signal_Limit/_minval: Value=KOUTP_USSStaRCR_flg_minval
      link override Signal_Override/_ovrdflg: Value=KOUTP_USSStaRCR_flg_ovrdflg
      link override Signal_Override/_ovrdval: Value=KOUTP_USSStaRCR_flg_ovrdval
  VAPM_USSStaRLL_flg_Inproc : FVT_lib/outp/OverrideAndLimit  SystemSampleTime=-1  VariantActivationTime=update diagram  Latency=0  AutoFrameSizeCalculation=off
      link override Signal_Limit/_maxval: Value=KOUTP_USSStaRLL_flg_maxval
      link override Signal_Limit/_minval: Value=KOUTP_USSStaRLL_flg_minval
      link override Signal_Override/_ovrdflg: Value=KOUTP_USSStaRLL_flg_ovrdflg
      link override Signal_Override/_ovrdval: Value=KOUTP_USSStaRLL_flg_ovrdval
  VAPM_USSStaRLR_flg_Inproc : FVT_lib/outp/OverrideAndLimit  SystemSampleTime=-1  VariantActivationTime=update diagram  Latency=0  AutoFrameSizeCalculation=off
      link override Signal_Limit/_maxval: Value=KOUTP_USSStaRLR_flg_maxval
      link override Signal_Limit/_minval: Value=KOUTP_USSStaRLR_flg_minval
      link override Signal_Override/_ovrdflg: Value=KOUTP_USSStaRLR_flg_ovrdflg
      link override Signal_Override/_ovrdval: Value=KOUTP_USSStaRLR_flg_ovrdval
  VAPM_USSStaRML_flg_Inproc : FVT_lib/outp/OverrideAndLimit  SystemSampleTime=-1  VariantActivationTime=update diagram  Latency=0  AutoFrameSizeCalculation=off
      link override Signal_Limit/_maxval: Value=KOUTP_USSStaRML_flg_maxval
      link override Signal_Limit/_minval: Value=KOUTP_USSStaRML_flg_minval
      link override Signal_Override/_ovrdflg: Value=KOUTP_USSStaRML_flg_ovrdflg
      link override Signal_Override/_ovrdval: Value=KOUTP_USSStaRML_flg_ovrdval
  VAPM_USSStaRMR_flg_Inproc : FVT_lib/outp/OverrideAndLimit  SystemSampleTime=-1  VariantActivationTime=update diagram  Latency=0  AutoFrameSizeCalculation=off
      link override Signal_Limit/_maxval: Value=KOUTP_USSStaRMR_flg_maxval
      link override Signal_Limit/_minval: Value=KOUTP_USSStaRMR_flg_minval
      link override Signal_Override/_ovrdflg: Value=KOUTP_USSStaRMR_flg_ovrdflg
      link override Signal_Override/_ovrdval: Value=KOUTP_USSStaRMR_flg_ovrdval
  VAPM_VehSpeedTimeOut_flg_Inproc : FVT_lib/outp/OverrideAndLimit  SystemSampleTime=-1  VariantActivationTime=update diagram  Latency=0  AutoFrameSizeCalculation=off
      link override Signal_Limit/_maxval: Value=KOUTP_VehSpeedTimeOut_flg_maxval
      link override Signal_Limit/_minval: Value=KOUTP_VehSpeedTimeOut_flg_minval
      link override Signal_Override/_ovrdflg: Value=KOUTP_VehSpeedTimeOut_flg_ovrdflg
      link override Signal_Override/_ovrdval: Value=KOUTP_VehSpeedTimeOut_flg_ovrdval
  VAPM_VehSpeed_kph_Inproc : FVT_lib/outp/OverrideAndLimit  SystemSampleTime=-1  VariantActivationTime=update diagram  Latency=0  AutoFrameSizeCalculation=off
      link override Signal_Limit/_maxval: Value=KOUTP_VehSpeed_kph_maxval
      link override Signal_Limit/_minval: Value=KOUTP_VehSpeed_kph_minval
      link override Signal_Override/_ovrdflg: Value=KOUTP_VehSpeed_kph_ovrdflg
      link override Signal_Override/_ovrdval: Value=KOUTP_VehSpeed_kph_ovrdval
  VAPM_YawRateTimeOut_flg_Inproc : FVT_lib/outp/OverrideAndLimit  SystemSampleTime=-1  VariantActivationTime=update diagram  Latency=0  AutoFrameSizeCalculation=off
      link override Signal_Limit/_maxval: Value=KOUTP_YawRateTimeOut_flg_maxval
      link override Signal_Limit/_minval: Value=KOUTP_YawRateTimeOut_flg_minval
      link override Signal_Override/_ovrdflg: Value=KOUTP_YawRateTimeOut_flg_ovrdflg
      link override Signal_Override/_ovrdval: Value=KOUTP_YawRateTimeOut_flg_ovrdval
  VAPM_YawRateVTimeOut_flg_Inproc : FVT_lib/outp/OverrideAndLimit  SystemSampleTime=-1  VariantActivationTime=update diagram  Latency=0  AutoFrameSizeCalculation=off
      link override Signal_Limit/_maxval: Value=KOUTP_YawRateVTimeOut_flg_maxval
      link override Signal_Limit/_minval: Value=KOUTP_YawRateVTimeOut_flg_minval
      link override Signal_Override/_ovrdflg: Value=KOUTP_YawRateVTimeOut_flg_ovrdflg
      link override Signal_Override/_ovrdval: Value=KOUTP_YawRateVTimeOut_flg_ovrdval
  VAPM_YawRateV_flg_Inproc : FVT_lib/outp/OverrideAndLimit  SystemSampleTime=-1  VariantActivationTime=update diagram  Latency=0  AutoFrameSizeCalculation=off
      link override Signal_Limit/_maxval: Value=KOUTP_YawRateV_flg_maxval
      link override Signal_Limit/_minval: Value=KOUTP_YawRateV_flg_minval
      link override Signal_Override/_ovrdflg: Value=KOUTP_YawRateV_flg_ovrdflg
      link override Signal_Override/_ovrdval: Value=KOUTP_YawRateV_flg_ovrdval
  VAPM_YawRate_degps_Inproc : FVT_lib/outp/OverrideAndLimit  SystemSampleTime=-1  VariantActivationTime=update diagram  Latency=0  AutoFrameSizeCalculation=off
      link override Signal_Limit/_maxval: Value=KOUTP_YawRate_degps_maxval
      link override Signal_Limit/_minval: Value=KOUTP_YawRate_degps_minval
      link override Signal_Override/_ovrdflg: Value=KOUTP_YawRate_degps_ovrdflg
      link override Signal_Override/_ovrdval: Value=KOUTP_YawRate_degps_ovrdval
  VBCM_APMDoorControlSta_flg_Inproc : FVT_lib/outp/OverrideAndLimit  SystemSampleTime=-1  VariantActivationTime=update diagram  Latency=0  AutoFrameSizeCalculation=off
      link override Signal_Limit/_maxval: Value=KOUTP_APMDoorControlSta_flg_maxval
      link override Signal_Limit/_minval: Value=KOUTP_APMDoorControlSta_flg_minval
      link override Signal_Override/_ovrdflg: Value=KOUTP_APMDoorControlSta_flg_ovrdflg
      link override Signal_Override/_ovrdval: Value=KOUTP_APMDoorControlSta_flg_ovrdval
  VBCM_APSOpenPTG_flg_Inproc : FVT_lib/outp/OverrideAndLimit  SystemSampleTime=-1  VariantActivationTime=update diagram  Latency=0  AutoFrameSizeCalculation=off
      link override Signal_Limit/_maxval: Value=KOUTP_APSOpenPTG_flg_maxval
      link override Signal_Limit/_minval: Value=KOUTP_APSOpenPTG_flg_minval
      link override Signal_Override/_ovrdflg: Value=KOUTP_APSOpenPTG_flg_ovrdflg
      link override Signal_Override/_ovrdval: Value=KOUTP_APSOpenPTG_flg_ovrdval
  VBCM_ATCtrl_enum_Inproc : FVT_lib/outp/OverrideAndLimit  SystemSampleTime=-1  VariantActivationTime=update diagram  Latency=0  AutoFrameSizeCalculation=off
      link override Signal_Limit/_maxval: Value=KOUTP_ATCtrl_enum_maxval
      link override Signal_Limit/_minval: Value=KOUTP_ATCtrl_enum_minval
      link override Signal_Override/_ovrdflg: Value=KOUTP_ATCtrl_enum_ovrdflg
      link override Signal_Override/_ovrdval: Value=KOUTP_ATCtrl_enum_ovrdval
  VBCM_AllDoorSW_flg_Inproc : FVT_lib/outp/OverrideAndLimit  SystemSampleTime=-1  VariantActivationTime=update diagram  Latency=0  AutoFrameSizeCalculation=off
      link override Signal_Limit/_maxval: Value=KOUTP_AllDoorSW_flg_maxval
      link override Signal_Limit/_minval: Value=KOUTP_AllDoorSW_flg_minval
      link override Signal_Override/_ovrdflg: Value=KOUTP_AllDoorSW_flg_ovrdflg
      link override Signal_Override/_ovrdval: Value=KOUTP_AllDoorSW_flg_ovrdval
  VBCM_AmbLightBreath1_flg_Inproc : FVT_lib/outp/OverrideAndLimit  SystemSampleTime=-1  VariantActivationTime=update diagram  Latency=0  AutoFrameSizeCalculation=off
      link override Signal_Limit/_maxval: Value=KOUTP_AmbLightBreath1_flg_maxval
      link override Signal_Limit/_minval: Value=KOUTP_AmbLightBreath1_flg_minval
      link override Signal_Override/_ovrdflg: Value=KOUTP_AmbLightBreath1_flg_ovrdflg
      link override Signal_Override/_ovrdval: Value=KOUTP_AmbLightBreath1_flg_ovrdval
  VBCM_AmbLightBreath2_flg_Inproc : FVT_lib/outp/OverrideAndLimit  SystemSampleTime=-1  VariantActivationTime=update diagram  Latency=0  AutoFrameSizeCalculation=off
      link override Signal_Limit/_maxval: Value=KOUTP_AmbLightBreath2_flg_maxval
      link override Signal_Limit/_minval: Value=KOUTP_AmbLightBreath2_flg_minval
      link override Signal_Override/_ovrdflg: Value=KOUTP_AmbLightBreath2_flg_ovrdflg
      link override Signal_Override/_ovrdval: Value=KOUTP_AmbLightBreath2_flg_ovrdval
  VBCM_AmbLightBreath3_flg_Inproc : FVT_lib/outp/OverrideAndLimit  SystemSampleTime=-1  VariantActivationTime=update diagram  Latency=0  AutoFrameSizeCalculation=off
      link override Signal_Limit/_maxval: Value=KOUTP_AmbLightBreath3_flg_maxval
      link override Signal_Limit/_minval: Value=KOUTP_AmbLightBreath3_flg_minval
      link override Signal_Override/_ovrdflg: Value=KOUTP_AmbLightBreath3_flg_ovrdflg
      link override Signal_Override/_ovrdval: Value=KOUTP_AmbLightBreath3_flg_ovrdval
  VBCM_AmbLightBrightness1_enum_Inproc : FVT_lib/outp/OverrideAndLimit  SystemSampleTime=-1  VariantActivationTime=update diagram  Latency=0  AutoFrameSizeCalculation=off
      link override Signal_Limit/_maxval: Value=KOUTP_AmbLightBrightness1_enum_maxval
      link override Signal_Limit/_minval: Value=KOUTP_AmbLightBrightness1_enum_minval
      link override Signal_Override/_ovrdflg: Value=KOUTP_AmbLightBrightness1_enum_ovrdflg
      link override Signal_Override/_ovrdval: Value=KOUTP_AmbLightBrightness1_enum_ovrdval
  VBCM_AmbLightBrightness2_enum_Inproc : FVT_lib/outp/OverrideAndLimit  SystemSampleTime=-1  VariantActivationTime=update diagram  Latency=0  AutoFrameSizeCalculation=off
      link override Signal_Limit/_maxval: Value=KOUTP_AmbLightBrightness2_enum_maxval
      link override Signal_Limit/_minval: Value=KOUTP_AmbLightBrightness2_enum_minval
      link override Signal_Override/_ovrdflg: Value=KOUTP_AmbLightBrightness2_enum_ovrdflg
      link override Signal_Override/_ovrdval: Value=KOUTP_AmbLightBrightness2_enum_ovrdval
  VBCM_AmbLightBrightness3_enum_Inproc : FVT_lib/outp/OverrideAndLimit  SystemSampleTime=-1  VariantActivationTime=update diagram  Latency=0  AutoFrameSizeCalculation=off
      link override Signal_Limit/_maxval: Value=KOUTP_AmbLightBrightness3_enum_maxval
      link override Signal_Limit/_minval: Value=KOUTP_AmbLightBrightness3_enum_minval
      link override Signal_Override/_ovrdflg: Value=KOUTP_AmbLightBrightness3_enum_ovrdflg
      link override Signal_Override/_ovrdval: Value=KOUTP_AmbLightBrightness3_enum_ovrdval
  VBCM_AmbLightColor1_enum_Inproc : FVT_lib/outp/OverrideAndLimit  SystemSampleTime=-1  VariantActivationTime=update diagram  Latency=0  AutoFrameSizeCalculation=off
      link override Signal_Limit/_maxval: Value=KOUTP_AmbLightColor1_enum_maxval
      link override Signal_Limit/_minval: Value=KOUTP_AmbLightColor1_enum_minval
      link override Signal_Override/_ovrdflg: Value=KOUTP_AmbLightColor1_enum_ovrdflg
      link override Signal_Override/_ovrdval: Value=KOUTP_AmbLightColor1_enum_ovrdval
  VBCM_AmbLightColor2_enum_Inproc : FVT_lib/outp/OverrideAndLimit  SystemSampleTime=-1  VariantActivationTime=update diagram  Latency=0  AutoFrameSizeCalculation=off
      link override Signal_Limit/_maxval: Value=KOUTP_AmbLightColor2_enum_maxval
      link override Signal_Limit/_minval: Value=KOUTP_AmbLightColor2_enum_minval
      link override Signal_Override/_ovrdflg: Value=KOUTP_AmbLightColor2_enum_ovrdflg
      link override Signal_Override/_ovrdval: Value=KOUTP_AmbLightColor2_enum_ovrdval
  VBCM_AmbLightColor3_enum_Inproc : FVT_lib/outp/OverrideAndLimit  SystemSampleTime=-1  VariantActivationTime=update diagram  Latency=0  AutoFrameSizeCalculation=off
      link override Signal_Limit/_maxval: Value=KOUTP_AmbLightColor3_enum_maxval
      link override Signal_Limit/_minval: Value=KOUTP_AmbLightColor3_enum_minval
      link override Signal_Override/_ovrdflg: Value=KOUTP_AmbLightColor3_enum_ovrdflg
      link override Signal_Override/_ovrdval: Value=KOUTP_AmbLightColor3_enum_ovrdval
  VBCM_AntitheftSeatFlod_flg_Inproc : FVT_lib/outp/OverrideAndLimit  SystemSampleTime=-1  VariantActivationTime=update diagram  Latency=0  AutoFrameSizeCalculation=off
      link override Signal_Limit/_maxval: Value=KOUTP_AntitheftSeatFlod_flg_maxval
      link override Signal_Limit/_minval: Value=KOUTP_AntitheftSeatFlod_flg_minval
      link override Signal_Override/_ovrdflg: Value=KOUTP_AntitheftSeatFlod_flg_ovrdflg
      link override Signal_Override/_ovrdval: Value=KOUTP_AntitheftSeatFlod_flg_ovrdval
  VBCM_AntitheftSta_enum_Inproc : FVT_lib/outp/OverrideAndLimit  SystemSampleTime=-1  VariantActivationTime=update diagram  Latency=0  AutoFrameSizeCalculation=off
      link override Signal_Limit/_maxval: Value=KOUTP_AntitheftSta_enum_maxval
      link override Signal_Limit/_minval: Value=KOUTP_AntitheftSta_enum_minval
      link override Signal_Override/_ovrdflg: Value=KOUTP_AntitheftSta_enum_ovrdflg
      link override Signal_Override/_ovrdval: Value=KOUTP_AntitheftSta_enum_ovrdval
  VBCM_BCMBuzzerReq_flg_Inproc : FVT_lib/outp/OverrideAndLimit  SystemSampleTime=-1  VariantActivationTime=update diagram  Latency=0  AutoFrameSizeCalculation=off
      link override Signal_Limit/_maxval: Value=KOUTP_BCMBuzzerReq_flg_maxval
      link override Signal_Limit/_minval: Value=KOUTP_BCMBuzzerReq_flg_minval
      link override Signal_Override/_ovrdflg: Value=KOUTP_BCMBuzzerReq_flg_ovrdflg
      link override Signal_Override/_ovrdval: Value=KOUTP_BCMBuzzerReq_flg_ovrdval
  VBCM_BCMDoorLockSta_flg_Inproc : FVT_lib/outp/OverrideAndLimit  SystemSampleTime=-1  VariantActivationTime=update diagram  Latency=0  AutoFrameSizeCalculation=off
      link override Signal_Limit/_maxval: Value=KOUTP_BCMDoorLockSta_flg_maxval
      link override Signal_Limit/_minval: Value=KOUTP_BCMDoorLockSta_flg_minval
      link override Signal_Override/_ovrdflg: Value=KOUTP_BCMDoorLockSta_flg_ovrdflg
      link override Signal_Override/_ovrdval: Value=KOUTP_BCMDoorLockSta_flg_ovrdval
  VBCM_BrakeLamp_flg_Inproc : FVT_lib/outp/OverrideAndLimit  SystemSampleTime=-1  VariantActivationTime=update diagram  Latency=0  AutoFrameSizeCalculation=off
      link override Signal_Limit/_maxval: Value=KOUTP_BrakeLamp_flg_maxval
      link override Signal_Limit/_minval: Value=KOUTP_BrakeLamp_flg_minval
      link override Signal_Override/_ovrdflg: Value=KOUTP_BrakeLamp_flg_ovrdflg
      link override Signal_Override/_ovrdval: Value=KOUTP_BrakeLamp_flg_ovrdval
  VBCM_CTDCtrl_enum_Inproc : FVT_lib/outp/OverrideAndLimit  SystemSampleTime=-1  VariantActivationTime=update diagram  Latency=0  AutoFrameSizeCalculation=off
      link override Signal_Limit/_maxval: Value=KOUTP_CTDCtrl_enum_maxval
      link override Signal_Limit/_minval: Value=KOUTP_CTDCtrl_enum_minval
      link override Signal_Override/_ovrdflg: Value=KOUTP_CTDCtrl_enum_ovrdflg
      link override Signal_Override/_ovrdval: Value=KOUTP_CTDCtrl_enum_ovrdval
  VBCM_CTDLockSW_flg_Inproc : FVT_lib/outp/OverrideAndLimit  SystemSampleTime=-1  VariantActivationTime=update diagram  Latency=0  AutoFrameSizeCalculation=off
      link override Signal_Limit/_maxval: Value=KOUTP_CTDLockSW_flg_maxval
      link override Signal_Limit/_minval: Value=KOUTP_CTDLockSW_flg_minval
      link override Signal_Override/_ovrdflg: Value=KOUTP_CTDLockSW_flg_ovrdflg
      link override Signal_Override/_ovrdval: Value=KOUTP_CTDLockSW_flg_ovrdval
  VBCM_CountAlarm_enum_Inproc : FVT_lib/outp/OverrideAndLimit  SystemSampleTime=-1  VariantActivationTime=update diagram  Latency=0  AutoFrameSizeCalculation=off
      link override Signal_Limit/_maxval: Value=KOUTP_CountAlarm_enum_maxval
      link override Signal_Limit/_minval: Value=KOUTP_CountAlarm_enum_minval
      link override Signal_Override/_ovrdflg: Value=KOUTP_CountAlarm_enum_ovrdflg
      link override Signal_Override/_ovrdval: Value=KOUTP_CountAlarm_enum_ovrdval
  VBCM_CrashDetd_flg_Inproc : FVT_lib/outp/OverrideAndLimit  SystemSampleTime=-1  VariantActivationTime=update diagram  Latency=0  AutoFrameSizeCalculation=off
      link override Signal_Limit/_maxval: Value=KOUTP_CrashDetd_flg_maxval
      link override Signal_Limit/_minval: Value=KOUTP_CrashDetd_flg_minval
      link override Signal_Override/_ovrdflg: Value=KOUTP_CrashDetd_flg_ovrdflg
      link override Signal_Override/_ovrdval: Value=KOUTP_CrashDetd_flg_ovrdval
  VBCM_DimmerEN_flg_Inproc : FVT_lib/outp/OverrideAndLimit  SystemSampleTime=-1  VariantActivationTime=update diagram  Latency=0  AutoFrameSizeCalculation=off
      link override Signal_Limit/_maxval: Value=KOUTP_DimmerEN_flg_maxval
      link override Signal_Limit/_minval: Value=KOUTP_DimmerEN_flg_minval
      link override Signal_Override/_ovrdflg: Value=KOUTP_DimmerEN_flg_ovrdflg
      link override Signal_Override/_ovrdval: Value=KOUTP_DimmerEN_flg_ovrdval
  VBCM_Dimmer_pct_Inproc : FVT_lib/outp/OverrideAndLimit  SystemSampleTime=-1  VariantActivationTime=update diagram  Latency=0  AutoFrameSizeCalculation=off
      link override Signal_Limit/_maxval: Value=KOUTP_Dimmer_pct_maxval
      link override Signal_Limit/_minval: Value=KOUTP_Dimmer_pct_minval
      link override Signal_Override/_ovrdflg: Value=KOUTP_Dimmer_pct_ovrdflg
      link override Signal_Override/_ovrdval: Value=KOUTP_Dimmer_pct_ovrdval
  VBCM_DoorLockIND_flg_Inproc : FVT_lib/outp/OverrideAndLimit  SystemSampleTime=-1  VariantActivationTime=update diagram  Latency=0  AutoFrameSizeCalculation=off
      link override Signal_Limit/_maxval: Value=KOUTP_DoorLockIND_flg_maxval
      link override Signal_Limit/_minval: Value=KOUTP_DoorLockIND_flg_minval
      link override Signal_Override/_ovrdflg: Value=KOUTP_DoorLockIND_flg_ovrdflg
      link override Signal_Override/_ovrdval: Value=KOUTP_DoorLockIND_flg_ovrdval
  VBCM_DrDoorSW_flg_Inproc : FVT_lib/outp/OverrideAndLimit  SystemSampleTime=-1  VariantActivationTime=update diagram  Latency=0  AutoFrameSizeCalculation=off
      link override Signal_Limit/_maxval: Value=KOUTP_DrDoorSW_flg_maxval
      link override Signal_Limit/_minval: Value=KOUTP_DrDoorSW_flg_minval
      link override Signal_Override/_ovrdflg: Value=KOUTP_DrDoorSW_flg_ovrdflg
      link override Signal_Override/_ovrdval: Value=KOUTP_DrDoorSW_flg_ovrdval
  VBCM_FollowMe_flg_Inproc : FVT_lib/outp/OverrideAndLimit  SystemSampleTime=-1  VariantActivationTime=update diagram  Latency=0  AutoFrameSizeCalculation=off
      link override Signal_Limit/_maxval: Value=KOUTP_FollowMe_flg_maxval
      link override Signal_Limit/_minval: Value=KOUTP_FollowMe_flg_minval
      link override Signal_Override/_ovrdflg: Value=KOUTP_FollowMe_flg_ovrdflg
      link override Signal_Override/_ovrdval: Value=KOUTP_FollowMe_flg_ovrdval
  VBCM_FrChargingDoorCtrl_enum_Inproc : FVT_lib/outp/OverrideAndLimit  SystemSampleTime=-1  VariantActivationTime=update diagram  Latency=0  AutoFrameSizeCalculation=off
      link override Signal_Limit/_maxval: Value=KOUTP_FrChargingDoorCtrl_enum_maxval
      link override Signal_Limit/_minval: Value=KOUTP_FrChargingDoorCtrl_enum_minval
      link override Signal_Override/_ovrdflg: Value=KOUTP_FrChargingDoorCtrl_enum_ovrdflg
      link override Signal_Override/_ovrdval: Value=KOUTP_FrChargingDoorCtrl_enum_ovrdval
  VBCM_FrWiperH_flg_Inproc : FVT_lib/outp/OverrideAndLimit  SystemSampleTime=-1  VariantActivationTime=update diagram  Latency=0  AutoFrameSizeCalculation=off
      link override Signal_Limit/_maxval: Value=KOUTP_FrWiperH_flg_maxval
      link override Signal_Limit/_minval: Value=KOUTP_FrWiperH_flg_minval
      link override Signal_Override/_ovrdflg: Value=KOUTP_FrWiperH_flg_ovrdflg
      link override Signal_Override/_ovrdval: Value=KOUTP_FrWiperH_flg_ovrdval
  VBCM_FrWiperL_flg_Inproc : FVT_lib/outp/OverrideAndLimit  SystemSampleTime=-1  VariantActivationTime=update diagram  Latency=0  AutoFrameSizeCalculation=off
      link override Signal_Limit/_maxval: Value=KOUTP_FrWiperL_flg_maxval
      link override Signal_Limit/_minval: Value=KOUTP_FrWiperL_flg_minval
      link override Signal_Override/_ovrdflg: Value=KOUTP_FrWiperL_flg_ovrdflg
      link override Signal_Override/_ovrdval: Value=KOUTP_FrWiperL_flg_ovrdval
  VBCM_FuelDoorPos_flg_Inproc : FVT_lib/outp/OverrideAndLimit  SystemSampleTime=-1  VariantActivationTime=update diagram  Latency=0  AutoFrameSizeCalculation=off
      link override Signal_Limit/_maxval: Value=KOUTP_FuelDoorPos_flg_maxval
      link override Signal_Limit/_minval: Value=KOUTP_FuelDoorPos_flg_minval
      link override Signal_Override/_ovrdflg: Value=KOUTP_FuelDoorPos_flg_ovrdflg
      link override Signal_Override/_ovrdval: Value=KOUTP_FuelDoorPos_flg_ovrdval
  VBCM_HBeam_flg_Inproc : FVT_lib/outp/OverrideAndLimit  SystemSampleTime=-1  VariantActivationTime=update diagram  Latency=0  AutoFrameSizeCalculation=off
      link override Signal_Limit/_maxval: Value=KOUTP_HBeam_flg_maxval
      link override Signal_Limit/_minval: Value=KOUTP_HBeam_flg_minval
      link override Signal_Override/_ovrdflg: Value=KOUTP_HBeam_flg_ovrdflg
      link override Signal_Override/_ovrdval: Value=KOUTP_HBeam_flg_ovrdval
  VBCM_HazardSW_flg_Inproc : FVT_lib/outp/OverrideAndLimit  SystemSampleTime=-1  VariantActivationTime=update diagram  Latency=0  AutoFrameSizeCalculation=off
      link override Signal_Limit/_maxval: Value=KOUTP_HazardSW_flg_maxval
      link override Signal_Limit/_minval: Value=KOUTP_HazardSW_flg_minval
      link override Signal_Override/_ovrdflg: Value=KOUTP_HazardSW_flg_ovrdflg
      link override Signal_Override/_ovrdval: Value=KOUTP_HazardSW_flg_ovrdval
  VBCM_HoodSW_flg_Inproc : FVT_lib/outp/OverrideAndLimit  SystemSampleTime=-1  VariantActivationTime=update diagram  Latency=0  AutoFrameSizeCalculation=off
      link override Signal_Limit/_maxval: Value=KOUTP_HoodSW_flg_maxval
      link override Signal_Limit/_minval: Value=KOUTP_HoodSW_flg_minval
      link override Signal_Override/_ovrdflg: Value=KOUTP_HoodSW_flg_ovrdflg
      link override Signal_Override/_ovrdval: Value=KOUTP_HoodSW_flg_ovrdval
  VBCM_HornCtrl_flg_Inproc : FVT_lib/outp/OverrideAndLimit  SystemSampleTime=-1  VariantActivationTime=update diagram  Latency=0  AutoFrameSizeCalculation=off
      link override Signal_Limit/_maxval: Value=KOUTP_HornCtrl_flg_maxval
      link override Signal_Limit/_minval: Value=KOUTP_HornCtrl_flg_minval
      link override Signal_Override/_ovrdflg: Value=KOUTP_HornCtrl_flg_ovrdflg
      link override Signal_Override/_ovrdval: Value=KOUTP_HornCtrl_flg_ovrdval
  VBCM_IVIPTGUSStaSW_flg_Inproc : FVT_lib/outp/OverrideAndLimit  SystemSampleTime=-1  VariantActivationTime=update diagram  Latency=0  AutoFrameSizeCalculation=off
      link override Signal_Limit/_maxval: Value=KOUTP_IVIPTGUSStaSW_flg_maxval
      link override Signal_Limit/_minval: Value=KOUTP_IVIPTGUSStaSW_flg_minval
      link override Signal_Override/_ovrdflg: Value=KOUTP_IVIPTGUSStaSW_flg_ovrdflg
      link override Signal_Override/_ovrdval: Value=KOUTP_IVIPTGUSStaSW_flg_ovrdval
  VBCM_IVIRST_flg_Inproc : FVT_lib/outp/OverrideAndLimit  SystemSampleTime=-1  VariantActivationTime=update diagram  Latency=0  AutoFrameSizeCalculation=off
      link override Signal_Limit/_maxval: Value=KOUTP_IVIRST_flg_maxval
      link override Signal_Limit/_minval: Value=KOUTP_IVIRST_flg_minval
      link override Signal_Override/_ovrdflg: Value=KOUTP_IVIRST_flg_ovrdflg
      link override Signal_Override/_ovrdval: Value=KOUTP_IVIRST_flg_ovrdval
  VBCM_LBSD_flg_Inproc : FVT_lib/outp/OverrideAndLimit  SystemSampleTime=-1  VariantActivationTime=update diagram  Latency=0  AutoFrameSizeCalculation=off
      link override Signal_Limit/_maxval: Value=KOUTP_LBSD_flg_maxval
      link override Signal_Limit/_minval: Value=KOUTP_LBSD_flg_minval
      link override Signal_Override/_ovrdflg: Value=KOUTP_LBSD_flg_ovrdflg
      link override Signal_Override/_ovrdval: Value=KOUTP_LBSD_flg_ovrdval
  VBCM_LBeam_flg_Inproc : FVT_lib/outp/OverrideAndLimit  SystemSampleTime=-1  VariantActivationTime=update diagram  Latency=0  AutoFrameSizeCalculation=off
      link override Signal_Limit/_maxval: Value=KOUTP_LBeam_flg_maxval
      link override Signal_Limit/_minval: Value=KOUTP_LBeam_flg_minval
      link override Signal_Override/_ovrdflg: Value=KOUTP_LBeam_flg_ovrdflg
      link override Signal_Override/_ovrdval: Value=KOUTP_LBeam_flg_ovrdval
  VBCM_LDRL_flg_Inproc : FVT_lib/outp/OverrideAndLimit  SystemSampleTime=-1  VariantActivationTime=update diagram  Latency=0  AutoFrameSizeCalculation=off
      link override Signal_Limit/_maxval: Value=KOUTP_LDRL_flg_maxval
      link override Signal_Limit/_minval: Value=KOUTP_LDRL_flg_minval
      link override Signal_Override/_ovrdflg: Value=KOUTP_LDRL_flg_ovrdflg
      link override Signal_Override/_ovrdval: Value=KOUTP_LDRL_flg_ovrdval
  VBCM_LDrvCtrlCmd_pct_Inproc : FVT_lib/outp/OverrideAndLimit  SystemSampleTime=-1  VariantActivationTime=update diagram  Latency=0  AutoFrameSizeCalculation=off
      link override Signal_Limit/_maxval: Value=KOUTP_LDrvCtrlCmd_pct_maxval
      link override Signal_Limit/_minval: Value=KOUTP_LDrvCtrlCmd_pct_minval
      link override Signal_Override/_ovrdflg: Value=KOUTP_LDrvCtrlCmd_pct_ovrdflg
      link override Signal_Override/_ovrdval: Value=KOUTP_LDrvCtrlCmd_pct_ovrdval
  VBCM_LPasCtrlCmd_pct_Inproc : FVT_lib/outp/OverrideAndLimit  SystemSampleTime=-1  VariantActivationTime=update diagram  Latency=0  AutoFrameSizeCalculation=off
      link override Signal_Limit/_maxval: Value=KOUTP_LPasCtrlCmd_pct_maxval
      link override Signal_Limit/_minval: Value=KOUTP_LPasCtrlCmd_pct_minval
      link override Signal_Override/_ovrdflg: Value=KOUTP_LPasCtrlCmd_pct_ovrdflg
      link override Signal_Override/_ovrdval: Value=KOUTP_LPasCtrlCmd_pct_ovrdval
  VBCM_LRLDCtrlCmd_pct_Inproc : FVT_lib/outp/OverrideAndLimit  SystemSampleTime=-1  VariantActivationTime=update diagram  Latency=0  AutoFrameSizeCalculation=off
      link override Signal_Limit/_maxval: Value=KOUTP_LRLDCtrlCmd_pct_maxval
      link override Signal_Limit/_minval: Value=KOUTP_LRLDCtrlCmd_pct_minval
      link override Signal_Override/_ovrdflg: Value=KOUTP_LRLDCtrlCmd_pct_ovrdflg
      link override Signal_Override/_ovrdval: Value=KOUTP_LRLDCtrlCmd_pct_ovrdval
  VBCM_LRRDCtrlCmd_pct_Inproc : FVT_lib/outp/OverrideAndLimit  SystemSampleTime=-1  VariantActivationTime=update diagram  Latency=0  AutoFrameSizeCalculation=off
      link override Signal_Limit/_maxval: Value=KOUTP_LRRDCtrlCmd_pct_maxval
      link override Signal_Limit/_minval: Value=KOUTP_LRRDCtrlCmd_pct_minval
      link override Signal_Override/_ovrdflg: Value=KOUTP_LRRDCtrlCmd_pct_ovrdflg
      link override Signal_Override/_ovrdval: Value=KOUTP_LRRDCtrlCmd_pct_ovrdval
  VBCM_LTurnLP_flg_Inproc : FVT_lib/outp/OverrideAndLimit  SystemSampleTime=-1  VariantActivationTime=update diagram  Latency=0  AutoFrameSizeCalculation=off
      link override Signal_Limit/_maxval: Value=KOUTP_LTurnLP_flg_maxval
      link override Signal_Limit/_minval: Value=KOUTP_LTurnLP_flg_minval
      link override Signal_Override/_ovrdflg: Value=KOUTP_LTurnLP_flg_ovrdflg
      link override Signal_Override/_ovrdval: Value=KOUTP_LTurnLP_flg_ovrdval
  VBCM_LampPwr_flg_Inproc : FVT_lib/outp/OverrideAndLimit  SystemSampleTime=-1  VariantActivationTime=update diagram  Latency=0  AutoFrameSizeCalculation=off
      link override Signal_Limit/_maxval: Value=KOUTP_LampPwr_flg_maxval
      link override Signal_Limit/_minval: Value=KOUTP_LampPwr_flg_minval
      link override Signal_Override/_ovrdflg: Value=KOUTP_LampPwr_flg_ovrdflg
      link override Signal_Override/_ovrdval: Value=KOUTP_LampPwr_flg_ovrdval
  VBCM_LockAlarm_enum_Inproc : FVT_lib/outp/OverrideAndLimit  SystemSampleTime=-1  VariantActivationTime=update diagram  Latency=0  AutoFrameSizeCalculation=off
      link override Signal_Limit/_maxval: Value=KOUTP_LockAlarm_enum_maxval
      link override Signal_Limit/_minval: Value=KOUTP_LockAlarm_enum_minval
      link override Signal_Override/_ovrdflg: Value=KOUTP_LockAlarm_enum_ovrdflg
      link override Signal_Override/_ovrdval: Value=KOUTP_LockAlarm_enum_ovrdval
  VBCM_LockSetting_flg_Inproc : FVT_lib/outp/OverrideAndLimit  SystemSampleTime=-1  VariantActivationTime=update diagram  Latency=0  AutoFrameSizeCalculation=off
      link override Signal_Limit/_maxval: Value=KOUTP_LockSetting_flg_maxval
      link override Signal_Limit/_minval: Value=KOUTP_LockSetting_flg_minval
      link override Signal_Override/_ovrdflg: Value=KOUTP_LockSetting_flg_ovrdflg
      link override Signal_Override/_ovrdval: Value=KOUTP_LockSetting_flg_ovrdval
  VBCM_MFRDNBrightReq_pct_Inproc : FVT_lib/outp/OverrideAndLimit  SystemSampleTime=-1  VariantActivationTime=update diagram  Latency=0  AutoFrameSizeCalculation=off
      link override Signal_Limit/_maxval: Value=KOUTP_MFRDNBrightReq_pct_maxval
      link override Signal_Limit/_minval: Value=KOUTP_MFRDNBrightReq_pct_minval
      link override Signal_Override/_ovrdflg: Value=KOUTP_MFRDNBrightReq_pct_ovrdflg
      link override Signal_Override/_ovrdval: Value=KOUTP_MFRDNBrightReq_pct_ovrdval
  VBCM_MFSWTri_flg_Inproc : FVT_lib/outp/OverrideAndLimit  SystemSampleTime=-1  VariantActivationTime=update diagram  Latency=0  AutoFrameSizeCalculation=off
      link override Signal_Limit/_maxval: Value=KOUTP_MFSWTri_flg_maxval
      link override Signal_Limit/_minval: Value=KOUTP_MFSWTri_flg_minval
      link override Signal_Override/_ovrdflg: Value=KOUTP_MFSWTri_flg_ovrdflg
      link override Signal_Override/_ovrdval: Value=KOUTP_MFSWTri_flg_ovrdval
  VBCM_MirrorCtrl_enum_Inproc : FVT_lib/outp/OverrideAndLimit  SystemSampleTime=-1  VariantActivationTime=update diagram  Latency=0  AutoFrameSizeCalculation=off
      link override Signal_Limit/_maxval: Value=KOUTP_MirrorCtrl_enum_maxval
      link override Signal_Limit/_minval: Value=KOUTP_MirrorCtrl_enum_minval
      link override Signal_Override/_ovrdflg: Value=KOUTP_MirrorCtrl_enum_ovrdflg
      link override Signal_Override/_ovrdval: Value=KOUTP_MirrorCtrl_enum_ovrdval
  VBCM_MirrorDefog_flg_Inproc : FVT_lib/outp/OverrideAndLimit  SystemSampleTime=-1  VariantActivationTime=update diagram  Latency=0  AutoFrameSizeCalculation=off
      link override Signal_Limit/_maxval: Value=KOUTP_MirrorDefog_flg_maxval
      link override Signal_Limit/_minval: Value=KOUTP_MirrorDefog_flg_minval
      link override Signal_Override/_ovrdflg: Value=KOUTP_MirrorDefog_flg_ovrdflg
      link override Signal_Override/_ovrdval: Value=KOUTP_MirrorDefog_flg_ovrdval
